simulink model "s_c856m4k_pre_buf"  (R2016b)
(part 3 of 50)

      mask TypeOptions io_dir: To Processor | From Processor
      mask Callback io_dir:
      | mask_enables = get_param(gcb, 'MaskEnables');
      | mask_names = get_param(gcb, 'MaskNames');
      | if strcmp(get_param(gcb, 'io_dir'), 'To Processor'),
      |     mask_enables{ismember(mask_names, 'sample_period')} = 'off';
      | else
      |     mask_enables{ismember(mask_names, 'sample_period')} = 'on';
      | end
      | set_param(gcb, 'MaskEnables', mask_enables);
  spead_valid_err_less : Subsystem  Tag=xps:sw_reg  AncestorBlock=xps_library/software_register  mask(swreg){io_dir=To Processor, io_delay=0, sample_period=1, names=reg, bitwidths=1, bin_pts=0, arith_types=2, sim_port=off, show_format=on}
      mask prompts: io_dir "I/O direction"; io_delay "I/O delay"; sample_period "Sample period"; names "Bitfield names [msb...lsb]"; bitwidths "Bitfield widths"; bin_pts "Bitfield binary pts"; arith_types "Bitfield types, ufix=0, fix=1, bool=2"; sim_port "Provide sim input/output?"; show_format "Print format string?"
      mask help: A 32-bit software-accessible register. Can be divided into bitfields of varying widths and types using the fields in the block mask.
      mask init:
      | swreg_init(gcb)
      settings: AttributesFormatString=1output:b = 1 bits
      mask TypeOptions io_dir: To Processor | From Processor
      mask Callback io_dir:
      | mask_enables = get_param(gcb, 'MaskEnables');
      | mask_names = get_param(gcb, 'MaskNames');
      | if strcmp(get_param(gcb, 'io_dir'), 'To Processor'),
      |     mask_enables{ismember(mask_names, 'sample_period')} = 'off';
      | else
      |     mask_enables{ismember(mask_names, 'sample_period')} = 'on';
      | end
      | set_param(gcb, 'MaskEnables', mask_enables);
  spead_valid_len : Subsystem  Tag=xps:sw_reg  AncestorBlock=xps_library/software_register  mask(swreg){io_dir=To Processor, io_delay=0, sample_period=1, names=reg, bitwidths=1, bin_pts=0, arith_types=2, sim_port=off, show_format=on}
      mask prompts: io_dir "I/O direction"; io_delay "I/O delay"; sample_period "Sample period"; names "Bitfield names [msb...lsb]"; bitwidths "Bitfield widths"; bin_pts "Bitfield binary pts"; arith_types "Bitfield types, ufix=0, fix=1, bool=2"; sim_port "Provide sim input/output?"; show_format "Print format string?"
      mask help: A 32-bit software-accessible register. Can be divided into bitfields of varying widths and types using the fields in the block mask.
      mask init:
      | swreg_init(gcb)
      settings: AttributesFormatString=1output:b = 1 bits
      mask TypeOptions io_dir: To Processor | From Processor
      mask Callback io_dir:
      | mask_enables = get_param(gcb, 'MaskEnables');
      | mask_names = get_param(gcb, 'MaskNames');
      | if strcmp(get_param(gcb, 'io_dir'), 'To Processor'),
      |     mask_enables{ismember(mask_names, 'sample_period')} = 'off';
      | else
      |     mask_enables{ismember(mask_names, 'sample_period')} = 'on';
      | end
      | set_param(gcb, 'MaskEnables', mask_enables);
  spead_valid_len_cnt : Subsystem  Tag=xps:sw_reg  AncestorBlock=xps_library/software_register  mask(swreg){io_dir=To Processor, io_delay=0, sample_period=1, names=reg, bitwidths=32, bin_pts=0, arith_types=0, sim_port=off, show_format=on}
      mask prompts: io_dir "I/O direction"; io_delay "I/O delay"; sample_period "Sample period"; names "Bitfield names [msb...lsb]"; bitwidths "Bitfield widths"; bin_pts "Bitfield binary pts"; arith_types "Bitfield types, ufix=0, fix=1, bool=2"; sim_port "Provide sim input/output?"; show_format "Print format string?"
      mask help: A 32-bit software-accessible register. Can be divided into bitfields of varying widths and types using the fields in the block mask.
      mask init:
      | swreg_init(gcb)
      settings: AttributesFormatString=1output:uf32.0 = 32 bits
      mask TypeOptions io_dir: To Processor | From Processor
      mask Callback io_dir:
      | mask_enables = get_param(gcb, 'MaskEnables');
      | mask_names = get_param(gcb, 'MaskNames');
      | if strcmp(get_param(gcb, 'io_dir'), 'To Processor'),
      |     mask_enables{ismember(mask_names, 'sample_period')} = 'off';
      | else
      |     mask_enables{ismember(mask_names, 'sample_period')} = 'on';
      | end
      | set_param(gcb, 'MaskEnables', mask_enables);
  speadsnap_control : Subsystem  Tag=xps:sw_reg  AncestorBlock=xps_library/software_register  mask(swreg){io_dir=From Processor, io_delay=0, sample_period=1, names=[speadsnap_arm], bitwidths=1, bin_pts=0, arith_types=2, sim_port=off, show_format=on}
      mask prompts: io_dir "I/O direction"; io_delay "I/O delay"; sample_period "Sample period"; names "Bitfield names [msb...lsb]"; bitwidths "Bitfield widths"; bin_pts "Bitfield binary pts"; arith_types "Bitfield types, ufix=0, fix=1, bool=2"; sim_port "Provide sim input/output?"; show_format "Print format string?"
      mask help: A 32-bit software-accessible register. Can be divided into bitfields of varying widths and types using the fields in the block mask.
      mask init:
      | swreg_init(gcb)
      settings: AttributesFormatString=1input:b = 1 bits
      mask TypeOptions io_dir: To Processor | From Processor
      mask Callback io_dir:
      | mask_enables = get_param(gcb, 'MaskEnables');
      | mask_names = get_param(gcb, 'MaskNames');
      | if strcmp(get_param(gcb, 'io_dir'), 'To Processor'),
      |     mask_enables{ismember(mask_names, 'sample_period')} = 'off';
      | else
      |     mask_enables{ismember(mask_names, 'sample_period')} = 'on';
      | end
      | set_param(gcb, 'MaskEnables', mask_enables);
  speadtime0_offset : Subsystem  Tag=xps:sw_reg  AncestorBlock=xps_library/software_register  mask(swreg){io_dir=From Processor, io_delay=1, sample_period=1, names=speadtime_offset0, bitwidths=32, bin_pts=0, arith_types=0, sim_port=on, show_format=on}
      mask prompts: io_dir "I/O direction"; io_delay "I/O delay"; sample_period "Sample period"; names "Bitfield names [msb...lsb]"; bitwidths "Bitfield widths"; bin_pts "Bitfield binary pts"; arith_types "Bitfield types, ufix=0, fix=1, bool=2"; sim_port "Provide sim input/output?"; show_format "Print format string?"
      mask help: A 32-bit software-accessible register. Can be divided into bitfields of varying widths and types using the fields in the block mask.
      mask init:
      | swreg_init(gcb)
      settings: AttributesFormatString=1input:uf32.0 = 32 bits
      mask TypeOptions io_dir: To Processor | From Processor
      mask Callback io_dir:
      | mask_enables = get_param(gcb, 'MaskEnables');
      | mask_names = get_param(gcb, 'MaskNames');
      | if strcmp(get_param(gcb, 'io_dir'), 'To Processor'),
      |     mask_enables{ismember(mask_names, 'sample_period')} = 'off';
      | else
      |     mask_enables{ismember(mask_names, 'sample_period')} = 'on';
      | end
      | set_param(gcb, 'MaskEnables', mask_enables);
  speadtime1_offset : Subsystem  Tag=xps:sw_reg  AncestorBlock=xps_library/software_register  mask(swreg){io_dir=From Processor, io_delay=1, sample_period=1, names=speadtime_offset1, bitwidths=32, bin_pts=0, arith_types=0, sim_port=on, show_format=on}
      mask prompts: io_dir "I/O direction"; io_delay "I/O delay"; sample_period "Sample period"; names "Bitfield names [msb...lsb]"; bitwidths "Bitfield widths"; bin_pts "Bitfield binary pts"; arith_types "Bitfield types, ufix=0, fix=1, bool=2"; sim_port "Provide sim input/output?"; show_format "Print format string?"
      mask help: A 32-bit software-accessible register. Can be divided into bitfields of varying widths and types using the fields in the block mask.
      mask init:
      | swreg_init(gcb)
      settings: AttributesFormatString=1input:uf32.0 = 32 bits
      mask TypeOptions io_dir: To Processor | From Processor
      mask Callback io_dir:
      | mask_enables = get_param(gcb, 'MaskEnables');
      | mask_names = get_param(gcb, 'MaskNames');
      | if strcmp(get_param(gcb, 'io_dir'), 'To Processor'),
      |     mask_enables{ismember(mask_names, 'sample_period')} = 'off';
      | else
      |     mask_enables{ismember(mask_names, 'sample_period')} = 'on';
      | end
      | set_param(gcb, 'MaskEnables', mask_enables);
  src_sel_cntrl : Subsystem  Tag=xps:sw_reg  AncestorBlock=xps_library/software_register  mask(swreg){io_dir=From Processor, io_delay=1, sample_period=1, names=[src_sel_0 src_sel_1], bitwidths=[2 2], bin_pts=[0 0], arith_types=[0 0], sim_port=on, show_format=on}
      mask prompts: io_dir "I/O direction"; io_delay "I/O delay"; sample_period "Sample period"; names "Bitfield names [msb...lsb]"; bitwidths "Bitfield widths"; bin_pts "Bitfield binary pts"; arith_types "Bitfield types, ufix=0, fix=1, bool=2"; sim_port "Provide sim input/output?"; show_format "Print format string?"
      mask help: A 32-bit software-accessible register. Can be divided into bitfields of varying widths and types using the fields in the block mask.
      mask init:
      | swreg_init(gcb)
      settings: AttributesFormatString=2 inputs:uf2.0,uf2.0 = 4 bits
      mask TypeOptions io_dir: To Processor | From Processor
      mask Callback io_dir:
      | mask_enables = get_param(gcb, 'MaskEnables');
      | mask_names = get_param(gcb, 'MaskNames');
      | if strcmp(get_param(gcb, 'io_dir'), 'To Processor'),
      |     mask_enables{ismember(mask_names, 'sample_period')} = 'off';
      | else
      |     mask_enables{ismember(mask_names, 'sample_period')} = 'on';
      | end
      | set_param(gcb, 'MaskEnables', mask_enables);
  ss_cwg0 : Subsystem  Tag=casper:bitsnap  AncestorBlock=casper_library_scopes/bitfield snapshot  mask(bitsnap){io_names=[d0 d1 d2 d3 d4 d5 d6 d7 gpio_trig], io_widths=[10 10 10 10 10 10 10 10 1], io_bps=[9 9 9 9 9 9 9 9 0], io_types=[1 1 1 1 1 1 1 1 2], show_format=on, snap_storage=bram, snap_dram_dimm=2, snap_dram_clock=250, snap_nsamples=11, snap_data_width=128, snap_offset=on, snap_circap=off, snap_value=off, snap_use_dsp48=off, snap_delay=1, extra_names=[c d], extra_widths=[30 2], extra_bps=[0 0], extra_types=[0 0]}
      mask prompts: io_names "Names [msb...lsb]"; io_widths "Bitwidths [msb...lsb]"; io_bps "Binary pts [msb...lsb]"; io_types "Data types [msb...lsb], ufix=0, fix=1, bool=2"; show_format "Print format string?"; snap_storage "Storage medium"; snap_dram_dimm "DRAM dimm"; snap_dram_clock "DRAM clock rate"; snap_nsamples "Number of Samples (2^?)"; snap_data_width "Data width"; snap_offset "Start delay support"; snap_circap "Circular capture support"; snap_value "Extra value capture support"; snap_use_dsp48 "Use DSP48s to implement counters"; snap_delay "Pre-snapshot delay"; extra_names "Names [msb...lsb]"; extra_widths "Widths [msb...lsb]"; extra_bps "Binary pts [msb...lsb]"; extra_types "Data types [msb...lsb], ufix=0, fix=1, bool=2"
      mask help:
      | A wrapped snapshot block. Allows specification of inputs to a snapblock word so the toolflow can automatically set up the scope.
      | See documentation for snapshot for explanation of parameters.
      mask init:
      | bitsnap_init(gcb);
      settings: AttributesFormatString=|
      | snap(9):f10.9,f10.9,f10.9,f10.9,f10.9,f10.9,f10.9,f10.9,b = 81 bits\n128 wide, 2048 deep
      | debugID: 126004058
      mask TypeOptions snap_storage: bram | dram
      mask Callback snap_storage: bitsnap_callback();
      mask TypeOptions snap_dram_dimm: 1 | 2 | 3 | 4
      mask TypeOptions snap_dram_clock: 200 | 250 | 266 | 300 | 333
      mask TypeOptions snap_data_width: 8 | 16 | 32 | 64 | 128
      mask Callback snap_value: bitsnap_callback();
  ss_fifo_in : Subsystem  Tag=casper:bitsnap  AncestorBlock=casper_library_scopes/bitfield snapshot  mask(bitsnap){io_names=[d0 d1 d2 d3 d4 d5 d6 d7 gpio_trig], io_widths=[10 10 10 10 10 10 10 10 1], io_bps=[9 9 9 9 9 9 9 9 0], io_types=[1 1 1 1 1 1 1 1 2], show_format=on, snap_storage=bram, snap_dram_dimm=2, snap_dram_clock=250, snap_nsamples=11, snap_data_width=128, snap_offset=on, snap_circap=off, snap_value=off, snap_use_dsp48=off, snap_delay=1, extra_names=[c d], extra_widths=[30 2], extra_bps=[0 0], extra_types=[0 0]}
      mask prompts: io_names "Names [msb...lsb]"; io_widths "Bitwidths [msb...lsb]"; io_bps "Binary pts [msb...lsb]"; io_types "Data types [msb...lsb], ufix=0, fix=1, bool=2"; show_format "Print format string?"; snap_storage "Storage medium"; snap_dram_dimm "DRAM dimm"; snap_dram_clock "DRAM clock rate"; snap_nsamples "Number of Samples (2^?)"; snap_data_width "Data width"; snap_offset "Start delay support"; snap_circap "Circular capture support"; snap_value "Extra value capture support"; snap_use_dsp48 "Use DSP48s to implement counters"; snap_delay "Pre-snapshot delay"; extra_names "Names [msb...lsb]"; extra_widths "Widths [msb...lsb]"; extra_bps "Binary pts [msb...lsb]"; extra_types "Data types [msb...lsb], ufix=0, fix=1, bool=2"
      mask help:
      | A wrapped snapshot block. Allows specification of inputs to a snapblock word so the toolflow can automatically set up the scope.
      | See documentation for snapshot for explanation of parameters.
      mask init:
      | bitsnap_init(gcb);
      settings: AttributesFormatString=|
      | snap(9):f10.9,f10.9,f10.9,f10.9,f10.9,f10.9,f10.9,f10.9,b = 81 bits\n128 wide, 2048 deep
      | debugID: 107099023
      mask TypeOptions snap_storage: bram | dram
      mask Callback snap_storage: bitsnap_callback();
      mask TypeOptions snap_dram_dimm: 1 | 2 | 3 | 4
      mask TypeOptions snap_dram_clock: 200 | 250 | 266 | 300 | 333
      mask TypeOptions snap_data_width: 8 | 16 | 32 | 64 | 128
      mask Callback snap_value: bitsnap_callback();
  ss_localtime : Subsystem  Tag=casper:bitsnap  AncestorBlock=casper_library_scopes/bitfield snapshot  mask(bitsnap){io_names=time, io_widths=64, io_bps=0, io_types=0, show_format=on, snap_storage=bram, snap_dram_dimm=2, snap_dram_clock=250, snap_nsamples=11, snap_data_width=64, snap_offset=on, snap_circap=off, snap_value=off, snap_use_dsp48=off, snap_delay=1, extra_names=[c d], extra_widths=[30 2], extra_bps=[0 0], extra_types=[0 0]}
      mask prompts: io_names "Names [msb...lsb]"; io_widths "Bitwidths [msb...lsb]"; io_bps "Binary pts [msb...lsb]"; io_types "Data types [msb...lsb], ufix=0, fix=1, bool=2"; show_format "Print format string?"; snap_storage "Storage medium"; snap_dram_dimm "DRAM dimm"; snap_dram_clock "DRAM clock rate"; snap_nsamples "Number of Samples (2^?)"; snap_data_width "Data width"; snap_offset "Start delay support"; snap_circap "Circular capture support"; snap_value "Extra value capture support"; snap_use_dsp48 "Use DSP48s to implement counters"; snap_delay "Pre-snapshot delay"; extra_names "Names [msb...lsb]"; extra_widths "Widths [msb...lsb]"; extra_bps "Binary pts [msb...lsb]"; extra_types "Data types [msb...lsb], ufix=0, fix=1, bool=2"
      mask help:
      | A wrapped snapshot block. Allows specification of inputs to a snapblock word so the toolflow can automatically set up the scope.
      | See documentation for snapshot for explanation of parameters.
      mask init:
      | bitsnap_init(gcb);
      settings: AttributesFormatString=|
      | snap(1):uf64.0 = 64 bits\n64 wide, 2048 deep
      | debugID: 12399183
      mask TypeOptions snap_storage: bram | dram
      mask Callback snap_storage: bitsnap_callback();
      mask TypeOptions snap_dram_dimm: 1 | 2 | 3 | 4
      mask TypeOptions snap_dram_clock: 200 | 250 | 266 | 300 | 333
      mask TypeOptions snap_data_width: 8 | 16 | 32 | 64 | 128
      mask Callback snap_value: bitsnap_callback();
  ss_trig_time_lsw : Subsystem  Tag=xps:sw_reg  AncestorBlock=xps_library/software_register  mask(swreg){io_dir=From Processor, io_delay=1, sample_period=1, names=reg, bitwidths=32, bin_pts=0, arith_types=0, sim_port=on, show_format=on}
      mask prompts: io_dir "I/O direction"; io_delay "I/O delay"; sample_period "Sample period"; names "Bitfield names [msb...lsb]"; bitwidths "Bitfield widths"; bin_pts "Bitfield binary pts"; arith_types "Bitfield types, ufix=0, fix=1, bool=2"; sim_port "Provide sim input/output?"; show_format "Print format string?"
      mask help: A 32-bit software-accessible register. Can be divided into bitfields of varying widths and types using the fields in the block mask.
      mask init:
      | swreg_init(gcb)
      settings: AttributesFormatString=1input:uf32.0 = 32 bits
      mask TypeOptions io_dir: To Processor | From Processor
      mask Callback io_dir:
      | mask_enables = get_param(gcb, 'MaskEnables');
      | mask_names = get_param(gcb, 'MaskNames');
      | if strcmp(get_param(gcb, 'io_dir'), 'To Processor'),
      |     mask_enables{ismember(mask_names, 'sample_period')} = 'off';
      | else
      |     mask_enables{ismember(mask_names, 'sample_period')} = 'on';
      | end
      | set_param(gcb, 'MaskEnables', mask_enables);
  ss_trig_time_msw : Subsystem  Tag=xps:sw_reg  AncestorBlock=xps_library/software_register  mask(swreg){io_dir=From Processor, io_delay=1, sample_period=1, names=reg, bitwidths=32, bin_pts=0, arith_types=0, sim_port=on, show_format=on}
      mask prompts: io_dir "I/O direction"; io_delay "I/O delay"; sample_period "Sample period"; names "Bitfield names [msb...lsb]"; bitwidths "Bitfield widths"; bin_pts "Bitfield binary pts"; arith_types "Bitfield types, ufix=0, fix=1, bool=2"; sim_port "Provide sim input/output?"; show_format "Print format string?"
      mask help: A 32-bit software-accessible register. Can be divided into bitfields of varying widths and types using the fields in the block mask.
      mask init:
      | swreg_init(gcb)
      settings: AttributesFormatString=1input:uf32.0 = 32 bits
      mask TypeOptions io_dir: To Processor | From Processor
      mask Callback io_dir:
      | mask_enables = get_param(gcb, 'MaskEnables');
      | mask_names = get_param(gcb, 'MaskNames');
      | if strcmp(get_param(gcb, 'io_dir'), 'To Processor'),
      |     mask_enables{ismember(mask_names, 'sample_period')} = 'off';
      | else
      |     mask_enables{ismember(mask_names, 'sample_period')} = 'on';
      | end
      | set_param(gcb, 'MaskEnables', mask_enables);
  start_flag_lsw : Subsystem  Tag=xps:sw_reg  AncestorBlock=xps_library/software_register  mask(swreg){io_dir=From Processor, io_delay=1, sample_period=1, names=reg, bitwidths=32, bin_pts=0, arith_types=0, sim_port=on, show_format=on}
      mask prompts: io_dir "I/O direction"; io_delay "I/O delay"; sample_period "Sample period"; names "Bitfield names [msb...lsb]"; bitwidths "Bitfield widths"; bin_pts "Bitfield binary pts"; arith_types "Bitfield types, ufix=0, fix=1, bool=2"; sim_port "Provide sim input/output?"; show_format "Print format string?"
      mask help: A 32-bit software-accessible register. Can be divided into bitfields of varying widths and types using the fields in the block mask.
      mask init:
      | swreg_init(gcb)
      settings: AttributesFormatString=1input:uf32.0 = 32 bits
      mask TypeOptions io_dir: To Processor | From Processor
      mask Callback io_dir:
      | mask_enables = get_param(gcb, 'MaskEnables');
      | mask_names = get_param(gcb, 'MaskNames');
      | if strcmp(get_param(gcb, 'io_dir'), 'To Processor'),
      |     mask_enables{ismember(mask_names, 'sample_period')} = 'off';
      | else
      |     mask_enables{ismember(mask_names, 'sample_period')} = 'on';
      | end
      | set_param(gcb, 'MaskEnables', mask_enables);
  start_flag_msw : Subsystem  Tag=xps:sw_reg  AncestorBlock=xps_library/software_register  mask(swreg){io_dir=From Processor, io_delay=1, sample_period=1, names=reg, bitwidths=32, bin_pts=0, arith_types=0, sim_port=on, show_format=on}
      mask prompts: io_dir "I/O direction"; io_delay "I/O delay"; sample_period "Sample period"; names "Bitfield names [msb...lsb]"; bitwidths "Bitfield widths"; bin_pts "Bitfield binary pts"; arith_types "Bitfield types, ufix=0, fix=1, bool=2"; sim_port "Provide sim input/output?"; show_format "Print format string?"
      mask help: A 32-bit software-accessible register. Can be divided into bitfields of varying widths and types using the fields in the block mask.
      mask init:
      | swreg_init(gcb)
      settings: AttributesFormatString=1input:uf32.0 = 32 bits
      mask TypeOptions io_dir: To Processor | From Processor
      mask Callback io_dir:
      | mask_enables = get_param(gcb, 'MaskEnables');
      | mask_names = get_param(gcb, 'MaskNames');
      | if strcmp(get_param(gcb, 'io_dir'), 'To Processor'),
      |     mask_enables{ismember(mask_names, 'sample_period')} = 'off';
      | else
      |     mask_enables{ismember(mask_names, 'sample_period')} = 'on';
      | end
      | set_param(gcb, 'MaskEnables', mask_enables);
  start_load_time_lsw : Subsystem  Tag=xps:sw_reg  AncestorBlock=xps_library/software_register  mask(swreg){io_dir=From Processor, io_delay=1, sample_period=1, names=reg, bitwidths=32, bin_pts=0, arith_types=0, sim_port=on, show_format=on}
      mask prompts: io_dir "I/O direction"; io_delay "I/O delay"; sample_period "Sample period"; names "Bitfield names [msb...lsb]"; bitwidths "Bitfield widths"; bin_pts "Bitfield binary pts"; arith_types "Bitfield types, ufix=0, fix=1, bool=2"; sim_port "Provide sim input/output?"; show_format "Print format string?"
      mask help: A 32-bit software-accessible register. Can be divided into bitfields of varying widths and types using the fields in the block mask.
      mask init:
      | swreg_init(gcb)
      settings: AttributesFormatString=1input:uf32.0 = 32 bits
      mask TypeOptions io_dir: To Processor | From Processor
      mask Callback io_dir:
      | mask_enables = get_param(gcb, 'MaskEnables');
      | mask_names = get_param(gcb, 'MaskNames');
      | if strcmp(get_param(gcb, 'io_dir'), 'To Processor'),
      |     mask_enables{ismember(mask_names, 'sample_period')} = 'off';
      | else
      |     mask_enables{ismember(mask_names, 'sample_period')} = 'on';
      | end
      | set_param(gcb, 'MaskEnables', mask_enables);
  start_load_time_msw : Subsystem  Tag=xps:sw_reg  AncestorBlock=xps_library/software_register  mask(swreg){io_dir=From Processor, io_delay=1, sample_period=1, names=reg, bitwidths=32, bin_pts=0, arith_types=0, sim_port=on, show_format=on}
      mask prompts: io_dir "I/O direction"; io_delay "I/O delay"; sample_period "Sample period"; names "Bitfield names [msb...lsb]"; bitwidths "Bitfield widths"; bin_pts "Bitfield binary pts"; arith_types "Bitfield types, ufix=0, fix=1, bool=2"; sim_port "Provide sim input/output?"; show_format "Print format string?"
      mask help: A 32-bit software-accessible register. Can be divided into bitfields of varying widths and types using the fields in the block mask.
      mask init:
      | swreg_init(gcb)
      settings: AttributesFormatString=1input:uf32.0 = 32 bits
      mask TypeOptions io_dir: To Processor | From Processor
      mask Callback io_dir:
      | mask_enables = get_param(gcb, 'MaskEnables');
      | mask_names = get_param(gcb, 'MaskNames');
      | if strcmp(get_param(gcb, 'io_dir'), 'To Processor'),
      |     mask_enables{ismember(mask_names, 'sample_period')} = 'off';
      | else
      |     mask_enables{ismember(mask_names, 'sample_period')} = 'on';
      | end
      | set_param(gcb, 'MaskEnables', mask_enables);
  start_time_lsw : Subsystem  Tag=xps:sw_reg  AncestorBlock=xps_library/software_register  mask(swreg){io_dir=From Processor, io_delay=1, sample_period=1, names=reg, bitwidths=32, bin_pts=0, arith_types=0, sim_port=on, show_format=on}
      mask prompts: io_dir "I/O direction"; io_delay "I/O delay"; sample_period "Sample period"; names "Bitfield names [msb...lsb]"; bitwidths "Bitfield widths"; bin_pts "Bitfield binary pts"; arith_types "Bitfield types, ufix=0, fix=1, bool=2"; sim_port "Provide sim input/output?"; show_format "Print format string?"
      mask help: A 32-bit software-accessible register. Can be divided into bitfields of varying widths and types using the fields in the block mask.
      mask init:
      | swreg_init(gcb)
      settings: AttributesFormatString=1input:uf32.0 = 32 bits
      mask TypeOptions io_dir: To Processor | From Processor
      mask Callback io_dir:
      | mask_enables = get_param(gcb, 'MaskEnables');
      | mask_names = get_param(gcb, 'MaskNames');
      | if strcmp(get_param(gcb, 'io_dir'), 'To Processor'),
      |     mask_enables{ismember(mask_names, 'sample_period')} = 'off';
      | else
      |     mask_enables{ismember(mask_names, 'sample_period')} = 'on';
      | end
      | set_param(gcb, 'MaskEnables', mask_enables);
  start_time_msw : Subsystem  Tag=xps:sw_reg  AncestorBlock=xps_library/software_register  mask(swreg){io_dir=From Processor, io_delay=1, sample_period=1, names=reg, bitwidths=32, bin_pts=0, arith_types=0, sim_port=on, show_format=on}
      mask prompts: io_dir "I/O direction"; io_delay "I/O delay"; sample_period "Sample period"; names "Bitfield names [msb...lsb]"; bitwidths "Bitfield widths"; bin_pts "Bitfield binary pts"; arith_types "Bitfield types, ufix=0, fix=1, bool=2"; sim_port "Provide sim input/output?"; show_format "Print format string?"
      mask help: A 32-bit software-accessible register. Can be divided into bitfields of varying widths and types using the fields in the block mask.
      mask init:
      | swreg_init(gcb)
      settings: AttributesFormatString=1input:uf32.0 = 32 bits
      mask TypeOptions io_dir: To Processor | From Processor
      mask Callback io_dir:
      | mask_enables = get_param(gcb, 'MaskEnables');
      | mask_names = get_param(gcb, 'MaskNames');
      | if strcmp(get_param(gcb, 'io_dir'), 'To Processor'),
      |     mask_enables{ismember(mask_names, 'sample_period')} = 'off';
      | else
      |     mask_enables{ismember(mask_names, 'sample_period')} = 'on';
      | end
      | set_param(gcb, 'MaskEnables', mask_enables);
  status0 : Subsystem  Tag=xps:sw_reg  AncestorBlock=xps_library/software_register  mask(swreg){io_dir=To Processor, io_delay=0, sample_period=1, names=[led_up led_rx led_tx tx_afull tx_overflow rx_overrun], bitwidths=1, bin_pts=0, arith_types=2, sim_port=off, show_format=on}
      mask prompts: io_dir "I/O direction"; io_delay "I/O delay"; sample_period "Sample period"; names "Bitfield names [msb...lsb]"; bitwidths "Bitfield widths"; bin_pts "Bitfield binary pts"; arith_types "Bitfield types, ufix=0, fix=1, bool=2"; sim_port "Provide sim input/output?"; show_format "Print format string?"
      mask help: A 32-bit software-accessible register. Can be divided into bitfields of varying widths and types using the fields in the block mask.
      mask init:
      | swreg_init(gcb)
      settings: AttributesFormatString=6 outputs:b,b,b,b,b,b = 6 bits
      mask TypeOptions io_dir: To Processor | From Processor
      mask Callback io_dir:
      | mask_enables = get_param(gcb, 'MaskEnables');
      | mask_names = get_param(gcb, 'MaskNames');
      | if strcmp(get_param(gcb, 'io_dir'), 'To Processor'),
      |     mask_enables{ismember(mask_names, 'sample_period')} = 'off';
      | else
      |     mask_enables{ismember(mask_names, 'sample_period')} = 'on';
      | end
      | set_param(gcb, 'MaskEnables', mask_enables);
  stop_load_time_lsw : Subsystem  Tag=xps:sw_reg  AncestorBlock=xps_library/software_register  mask(swreg){io_dir=From Processor, io_delay=1, sample_period=1, names=reg, bitwidths=32, bin_pts=0, arith_types=0, sim_port=on, show_format=on}
      mask prompts: io_dir "I/O direction"; io_delay "I/O delay"; sample_period "Sample period"; names "Bitfield names [msb...lsb]"; bitwidths "Bitfield widths"; bin_pts "Bitfield binary pts"; arith_types "Bitfield types, ufix=0, fix=1, bool=2"; sim_port "Provide sim input/output?"; show_format "Print format string?"
      mask help: A 32-bit software-accessible register. Can be divided into bitfields of varying widths and types using the fields in the block mask.
      mask init:
      | swreg_init(gcb)
      settings: AttributesFormatString=1input:uf32.0 = 32 bits
      mask TypeOptions io_dir: To Processor | From Processor
      mask Callback io_dir:
      | mask_enables = get_param(gcb, 'MaskEnables');
      | mask_names = get_param(gcb, 'MaskNames');
      | if strcmp(get_param(gcb, 'io_dir'), 'To Processor'),
      |     mask_enables{ismember(mask_names, 'sample_period')} = 'off';
      | else
      |     mask_enables{ismember(mask_names, 'sample_period')} = 'on';
      | end
      | set_param(gcb, 'MaskEnables', mask_enables);
  stop_load_time_msw : Subsystem  Tag=xps:sw_reg  AncestorBlock=xps_library/software_register  mask(swreg){io_dir=From Processor, io_delay=1, sample_period=1, names=reg, bitwidths=32, bin_pts=0, arith_types=0, sim_port=on, show_format=on}
      mask prompts: io_dir "I/O direction"; io_delay "I/O delay"; sample_period "Sample period"; names "Bitfield names [msb...lsb]"; bitwidths "Bitfield widths"; bin_pts "Bitfield binary pts"; arith_types "Bitfield types, ufix=0, fix=1, bool=2"; sim_port "Provide sim input/output?"; show_format "Print format string?"
      mask help: A 32-bit software-accessible register. Can be divided into bitfields of varying widths and types using the fields in the block mask.
      mask init:
      | swreg_init(gcb)
      settings: AttributesFormatString=1input:uf32.0 = 32 bits
      mask TypeOptions io_dir: To Processor | From Processor
      mask Callback io_dir:
      | mask_enables = get_param(gcb, 'MaskEnables');
      | mask_names = get_param(gcb, 'MaskNames');
      | if strcmp(get_param(gcb, 'io_dir'), 'To Processor'),
      |     mask_enables{ismember(mask_names, 'sample_period')} = 'off';
      | else
      |     mask_enables{ismember(mask_names, 'sample_period')} = 'on';
      | end
      | set_param(gcb, 'MaskEnables', mask_enables);
  test_control : Subsystem  Tag=xps:sw_reg  AncestorBlock=xps_library/software_register  mask(swreg){io_dir=From Processor, io_delay=0, sample_period=1, names=[sel_ramp80 rst_ramp80], bitwidths=1, bin_pts=0, arith_types=2, sim_port=on, show_format=on}
      mask prompts: io_dir "I/O direction"; io_delay "I/O delay"; sample_period "Sample period"; names "Bitfield names [msb...lsb]"; bitwidths "Bitfield widths"; bin_pts "Bitfield binary pts"; arith_types "Bitfield types, ufix=0, fix=1, bool=2"; sim_port "Provide sim input/output?"; show_format "Print format string?"
      mask help: A 32-bit software-accessible register. Can be divided into bitfields of varying widths and types using the fields in the block mask.
      mask init:
      | swreg_init(gcb)
      settings: AttributesFormatString=2 inputs:b,b = 2 bits
      mask TypeOptions io_dir: To Processor | From Processor
      mask Callback io_dir:
      | mask_enables = get_param(gcb, 'MaskEnables');
      | mask_names = get_param(gcb, 'MaskNames');
      | if strcmp(get_param(gcb, 'io_dir'), 'To Processor'),
      |     mask_enables{ismember(mask_names, 'sample_period')} = 'off';
      | else
      |     mask_enables{ismember(mask_names, 'sample_period')} = 'on';
      | end
      | set_param(gcb, 'MaskEnables', mask_enables);
  tick_offset_lsw : Subsystem  Tag=xps:sw_reg  AncestorBlock=xps_library/software_register  mask(swreg){io_dir=From Processor, io_delay=1, sample_period=1, names=reg, bitwidths=32, bin_pts=0, arith_types=0, sim_port=on, show_format=on}
      mask prompts: io_dir "I/O direction"; io_delay "I/O delay"; sample_period "Sample period"; names "Bitfield names [msb...lsb]"; bitwidths "Bitfield widths"; bin_pts "Bitfield binary pts"; arith_types "Bitfield types, ufix=0, fix=1, bool=2"; sim_port "Provide sim input/output?"; show_format "Print format string?"
      mask help: A 32-bit software-accessible register. Can be divided into bitfields of varying widths and types using the fields in the block mask.
      mask init:
      | swreg_init(gcb)
      settings: AttributesFormatString=1input:uf32.0 = 32 bits
      mask TypeOptions io_dir: To Processor | From Processor
      mask Callback io_dir:
      | mask_enables = get_param(gcb, 'MaskEnables');
      | mask_names = get_param(gcb, 'MaskNames');
      | if strcmp(get_param(gcb, 'io_dir'), 'To Processor'),
      |     mask_enables{ismember(mask_names, 'sample_period')} = 'off';
      | else
      |     mask_enables{ismember(mask_names, 'sample_period')} = 'on';
      | end
      | set_param(gcb, 'MaskEnables', mask_enables);
  tick_offset_msw : Subsystem  Tag=xps:sw_reg  AncestorBlock=xps_library/software_register  mask(swreg){io_dir=From Processor, io_delay=1, sample_period=1, names=reg, bitwidths=32, bin_pts=0, arith_types=0, sim_port=on, show_format=on}
      mask prompts: io_dir "I/O direction"; io_delay "I/O delay"; sample_period "Sample period"; names "Bitfield names [msb...lsb]"; bitwidths "Bitfield widths"; bin_pts "Bitfield binary pts"; arith_types "Bitfield types, ufix=0, fix=1, bool=2"; sim_port "Provide sim input/output?"; show_format "Print format string?"
      mask help: A 32-bit software-accessible register. Can be divided into bitfields of varying widths and types using the fields in the block mask.
      mask init:
      | swreg_init(gcb)
      settings: AttributesFormatString=1input:uf32.0 = 32 bits
      mask TypeOptions io_dir: To Processor | From Processor
      mask Callback io_dir:
      | mask_enables = get_param(gcb, 'MaskEnables');
      | mask_names = get_param(gcb, 'MaskNames');
      | if strcmp(get_param(gcb, 'io_dir'), 'To Processor'),
      |     mask_enables{ismember(mask_names, 'sample_period')} = 'off';
      | else
      |     mask_enables{ismember(mask_names, 'sample_period')} = 'on';
      | end
      | set_param(gcb, 'MaskEnables', mask_enables);
  ticks_since_mrst : Subsystem
  tvg_spead_time_with_pkt_ctr : Subsystem  mask{packetlen_bits=9}
      mask prompts: packetlen_bits "Packet length, num 80-bit words (2^?):"
  wng0 : Subsystem
  wng_corr : Subsystem
  wng_rst : Subsystem
  wr_addr{0..3} (4 alike) : xbsIndex_r4/Counter  cnt_type=Free Running  cnt_to=Inf  operation=Up  start_count=0  cnt_by_val=1  arith_type=Unsigned  n_bits=10  bin_pt=0  load_pin=off  rst=on  en=on  explicit_period=on  period=1  use_behavioral_HDL=off  implementation=Fabric  dbl_ovrd=off  block_type=counter
  tag scope: arb_en0=global, arb_rst0=global, cnt_rst=global, dram_addr_offset0=global, dram_rd_repeat0=global, dram_rd_repeat_delay0=global, dram_rd_trig0=global, dram_read_length0=global, dram_tvg0=global, dram_tvg_length0=global, local_time=global, tvg_sel0=global
  wires:
  gbe_porttx/1(in_reg) -> pipeline242/1(d)
  Constant197/1 -> gbe_porttx/1(sim_1)
  Constant75/1 -> gbe_iptx0/1(sim_1)
  Constant77/1 -> gbe_iptx1/1(sim_1)
  Constant78/1 -> gbe_iptx2/1(sim_1)
  Constant79/1 -> gbe_iptx3/1(sim_1)
  Constant80/1 -> digitiser_id/1(sim_1)
  Constant82/1 -> receptor_id/1(sim_1)
  Constant81/1 -> digitiser_id/2(sim_2)
  receptor_id/1(in_receptor_id) -> bus_create1/3(in3)
  Constant165/1 -> receptor_id/2(sim_2)
  Constant84/1 -> receptor_id/3(sim_3)
  [masked_time] -> Delay128/1
  tvg_spead_time_with_pkt_ctr/1(local_time) -> Delay131/1
  tvg_spead_time_with_pkt_ctr/3(tvg_data_pol0) -> Delay133/1
  tvg_spead_time_with_pkt_ctr/4(tvg_data_pol1) -> Delay134/1
  tvg_spead_time_with_pkt_ctr/2(spead_time) -> Delay132/1
  [fifoselect] -> edge_detect37/1(in), Inverter2/1
  Register5/1 -> [speadtime0]  "speadtime0"
  Inverter2/1 -> edge_detect38/1(in)
  edge_detect37/1(out) -> Register5/2
  edge_detect38/1(out) -> Register6/2
  Register6/1 -> [speadtime1]  "speadtime1"
  [mrst] -> ticks_since_mrst/1(reset)
  [sync] -> ticks_since_mrst/2(sync)
  ticks_since_mrst/1(time64) -> [local_time]  "localtime"
  [msync] -> [sync]  "sync"
  edge_detect20/1(out) -> [mrst]  "mrst"
  edge_detect6/1(out) -> [msync]  "msync"
  edge_detect36/1(out) -> Terminator83/1  "clr_status"
  [local_time] -> slice1/1, slice2/1
  Constant92/1 -> orig_control/3(sim_3)
  Constant149/1 -> orig_control/1(sim_1)
  Constant90/1 -> orig_control/2(sim_2)
  Constant98/1 -> orig_control/6(sim_6)
  Constant95/1 -> orig_control/5(sim_5)
  Constant124/1 -> orig_control/4(sim_4)
  Pulse Generator/1 -> orig_control/8(sim_8)
  [tick_offset] -> ticks_since_mrst/3(offset)
  edge_detect7/1(out) -> [load_tick_offset]  "mrst"
  Constant86/1 -> orig_control/9(sim_9)
  digitiser_id/1(in_digitiser_serial) -> bus_create1/1(in1)
  digitiser_id/2(in_digitiser_type) -> bus_create1/2(in2)
  Constant148/1 -> flag_setup/3(sim_3)
  Constant147/1 -> flag_setup/2(sim_2)
  Constant143/1 -> flag_setup/1(sim_1)
  Counter Free-Running3/1 -> Relational Operator4/2
  Constant152/1 -> Relational Operator4/1
  Relational Operator4/1 -> flag_setup/4(sim_4)
  Constant157/1 -> start_flag_msw/1(sim_1)
  Constant158/1 -> start_flag_lsw/1(sim_1)
  Constant156/1 -> end_flag_msw/1(sim_1)
  Constant155/1 -> end_flag_lsw/1(sim_1)
  Concat18/1 -> Delay83/1  "starttime"
  Concat19/1 -> Delay85/1  "stoptime"
  [flag_start_time] -> Delay80/1
  [local_time] -> Delay79/1, Delay81/1
  [flag_end_time] -> Delay82/1, Delay86/1
  Relational4/1 -> Logical24/2  "start_okay"
  [flag_armed] -> Delay78/1
  Relational5/1 -> Logical42/2  "end_okay"
  Logical24/1 -> Delay55/1  "start_okay"
  Logical42/1 -> Logical35/1  "end_okay"
  edge_detect41/1(out) -> [load_flag_time]  "loadtimes"
  Constant144/1 -> Register1/1
  edge_detect40/1(out) -> [reset_flag_time]  "rst"
  [reset_flag_time] -> Register1/2
  [load_flag_time] -> Register1/3
  Register1/1 -> [flag_armed]  "armed"
  Relational Operator3/1 -> flag_setup/5(sim_5)
  Relational8/1 -> Delay54/1  "zero_stop"
  Constant85/1 -> Relational8/2
  Logical35/1 -> Logical4/2  "eokay"
  Counter Free-Running2/1 -> Relational Operator3/2
  Constant154/1 -> Relational Operator3/1
  Logical43/1 -> sample_masking/2(den_in)
  Constant153/1 -> start_time_msw/1(sim_1)
  Constant159/1 -> start_time_lsw/1(sim_1)
  Constant94/1 -> end_time_msw/1(sim_1)
  Constant76/1 -> end_time_lsw/1(sim_1)
  Relational9/1 -> Logical44/2  "start_okay"
  Relational17/1 -> Logical46/2  "end_okay"
  [start_time] -> Delay72/1
  Relational19/1 -> Delay40/1  "first_sample"
  [end_time] -> Delay75/1
  Relational20/1 -> Delay41/1  "last_sample"
  [sample_end] -> sample_masking/6(sample_end)
  [sample_start] -> sample_masking/5(sample_start)
  sample_masking/2(den_out) -> Delay126/1  "enable"
  sample_masking/3(data_mask) -> Delay127/1  "mask"
  edge_detect11/1(out) -> [reset_en_time]  "reset_en_time"
  Relational Operator5/1 -> control_output/2(sim_2)
  Counter Free-Running4/1 -> Relational Operator6/2, Relational Operator5/2
  Constant142/1 -> Relational Operator5/1
  edge_detect12/1(out) -> [load_en_time]  "load_en_time"
  Concat10/1 -> Delay76/1
  Concat11/1 -> Delay77/1
  Constant88/1 -> Register2/1
  [reset_en_time] -> Register2/2
  [load_en_time] -> Register2/3
  Register2/1 -> [en_armed]  "armed"
  Logical44/1 -> Delay42/1  "start_okay"
  Logical46/1 -> Logical45/1  "end_okay"
  Logical45/1 -> Logical43/2
  Constant99/1 -> Delay70/1
  Relational18/1 -> Delay39/1
  Constant93/1 -> control_output/3(sim_3)
  Constant151/1 -> control_output/4(sim_4)
  Constant96/1 -> Relational Operator6/1
  Relational Operator6/1 -> control_output/1(sim_1)
  [data_enable] -> Delay129/1
  [sample_mask] -> Delay130/1
  Constant150/1 -> tick_offset_msw/1(sim_1)
  Constant176/1 -> tick_offset_lsw/1(sim_1)
  Concat16/1 -> Register3/1
  [load_tick_offset] -> Register3/2
  Register3/1 -> [tick_offset]
  wng0/1(bus_out) -> [wng0_tp0], pipeline443/1(d)
  bus_addsub/1(dout) -> Delay105/1
  bus_addsub2/1(dout) -> Delay95/1
  bus_addsub4/1(dout) -> bus_convert6/1(din)
  bus_mult/1(a*b) -> [cwg0_tp1], bus_convert/1(din)
  Constant123/1 -> scale_wng0/1(sim_1)
  Constant74/1 -> scale_wng_corr/1(sim_1)
  pipeline309/1(q) -> edge_detect12/1(in)
  pipeline320/1(q) -> edge_detect11/1(in)
  pipeline331/1(q) -> [sample_start]
  pipeline339/1(q) -> [sample_end]
  Delay76/1 -> [start_time]
  Delay77/1 -> [end_time]
  Delay83/1 -> [flag_start_time]
  Delay85/1 -> [flag_end_time]
  pipeline407/1(q) -> wng0/1(scale_16_14)
  pipeline206/1(q) -> [gbe_ip3]
  pipeline212/1(q) -> [gbe_ip2]
  pipeline220/1(q) -> [gbe_ip0]
  Delay126/1 -> [data_enable]
  Delay127/1 -> [sample_mask]
  Delay128/1 -> tvg_spead_time_with_pkt_ctr/1(localtime64)
  Delay129/1 -> tvg_spead_time_with_pkt_ctr/2(data_enable)
  Delay130/1 -> tvg_spead_time_with_pkt_ctr/3(data_mask)
  Delay131/1 -> [tvg_ltime]
  Delay132/1 -> [tvg_stime]
  Delay133/1 -> [tvg_pol0]
  Delay134/1 -> [tvg_pol1]
  Delay105/1 -> bus_convert2/1(din)
  Delay95/1 -> bus_convert4/1(din)
  Delay139/1 -> bus_addsub4/1(a)
  pipeline350/1(q) -> Concat10/1
  pipeline361/1(q) -> Concat10/2
  pipeline372/1(q) -> Concat11/1
  pipeline383/1(q) -> Concat11/2
  pipeline393/1(q) -> [hdr_0x3101]
  pipeline395/1(q) -> [pol0_id]
  pipeline396/1(q) -> [pol1_id]
  orig_control/1(in_up_cnt_rst) -> pipeline204/1(d)
  pipeline204/1(q) -> edge_detect31/1(in)
  orig_control/2(in_tvg_select0) -> pipeline205/1(d)
  orig_control/3(in_tvg_select1) -> pipeline297/1(d)
  orig_control/4(in_clr_status) -> pipeline394/1(d)
  orig_control/5(in_gbe_rst) -> pipeline405/1(d)
  orig_control/6(in_gbe_txen) -> pipeline416/1(d)
  orig_control/7(in_msync) -> pipeline424/1(d)
  orig_control/8(in_mrst) -> pipeline434/1(d)
  orig_control/9(in_load_tick_offset) -> pipeline445/1(d)
  pipeline445/1(q) -> edge_detect7/1(in)
  pipeline434/1(q) -> edge_detect20/1(in)
  pipeline424/1(q) -> edge_detect6/1(in)
  pipeline405/1(q) -> Terminator82/1
  pipeline394/1(q) -> edge_detect36/1(in)
  pipeline297/1(q) -> [tvg_select1]
  pipeline205/1(q) -> [tvg_select0]
  pipeline213/1(q) -> [gbe_ip1]
  gbe_iptx0/1(in_reg) -> pipeline220/1(d)
  gbe_iptx1/1(in_reg) -> pipeline213/1(d)
  gbe_iptx2/1(in_reg) -> pipeline212/1(d)
  gbe_iptx3/1(in_reg) -> pipeline206/1(d)
  tick_offset_msw/1(in_reg) -> pipeline264/1(d)
  pipeline264/1(q) -> Concat16/1
  tick_offset_lsw/1(in_reg) -> pipeline275/1(d)
  pipeline275/1(q) -> Concat16/2
  slice1/1 -> pipeline298/1(d)
  pipeline298/1(q) -> local_time_lsw1/1(out_reg)
  slice2/1 -> pipeline286/1(d)
  pipeline286/1(q) -> local_time_msw1/1(out_reg)
  end_time_lsw/1(in_reg) -> pipeline383/1(d)
  end_time_msw/1(in_reg) -> pipeline372/1(d)
  start_time_lsw/1(in_reg) -> pipeline361/1(d)
  start_time_msw/1(in_reg) -> pipeline350/1(d)
  control_output/4(in_sample_end) -> pipeline339/1(d)
  control_output/3(in_sample_start) -> pipeline331/1(d)
  control_output/2(in_reset_en_time) -> pipeline320/1(d)
  control_output/1(in_load_en_time) -> pipeline309/1(d)
  bus_create1/1(bus_out) -> pipeline393/1(d)
  receptor_id/2(in_pol0_id) -> pipeline395/1(d)
  receptor_id/3(in_pol1_id) -> pipeline396/1(d)
  flag_setup/1(in_adc_count) -> pipeline397/1(d)
  flag_setup/2(in_adc_flag) -> pipeline398/1(d)
  flag_setup/3(in_ndiode_flag) -> pipeline399/1(d)
  flag_setup/4(in_load_flags) -> pipeline400/1(d)
  flag_setup/5(in_reset_flags) -> pipeline401/1(d)
  pipeline401/1(q) -> edge_detect40/1(in)
  pipeline400/1(q) -> edge_detect41/1(in)
  pipeline399/1(q) -> [ndiode_flag]
  pipeline398/1(q) -> [adc_flag]
  pipeline397/1(q) -> [adc_count]
  start_flag_msw/1(in_reg) -> pipeline402/1(d)
  pipeline402/1(q) -> Concat18/1
  start_flag_lsw/1(in_reg) -> pipeline403/1(d)
  pipeline403/1(q) -> Concat18/2
  end_flag_msw/1(in_reg) -> pipeline404/1(d)
  pipeline404/1(q) -> Concat19/1
  end_flag_lsw/1(in_reg) -> pipeline406/1(d)
  pipeline406/1(q) -> Concat19/2
  pipeline418/1(q) -> bus_mult/2(b)
  pipeline443/1(q) -> bus_addsub/1(a)
  pipeline444/1(q) -> bus_addsub/2(b)
  wng_corr/1(bus_out) -> pipeline444/1(d)
  pipeline458/1(q) -> bus_addsub2/2(b)
  pipeline461/1(q) -> [cwg_80_1], [cwg_80_0]
  Delay46/1 -> bus_addsub4/2(b)
  Delay38/1 -> Logical46/1, Logical44/1
  Delay39/1 -> Logical45/2
  Delay40/1 -> Delay44/1
  Delay41/1 -> Delay45/1
  Delay42/1 -> Logical43/1
  Delay44/1 -> Delay47/1
  Delay45/1 -> Delay48/1
  Delay47/1 -> sample_masking/3(first_samples)
  Delay48/1 -> sample_masking/4(last_samples)
  Delay54/1 -> Logical35/2
  Delay55/1 -> Logical4/1
  Delay56/1 -> Delay57/1
  Delay57/1 -> Delay58/1
  Delay58/1 -> Delay59/1
  Delay59/1 -> sample_masking/1(timei)
  sample_masking/4(flag_valid) -> Delay60/1
  Delay60/1 -> [flag_en]
  Logical4/1 -> sample_masking/7(flag_en)  "flag_en"
  sample_masking/1(timeo) -> Delay61/1
  Delay61/1 -> [masked_time]
  [local_time] -> Delay63/1
  [en_armed] -> Delay64/1
  [local_time] -> Delay65/1, Delay67/1, Delay71/1, Delay74/1
  [start_time] -> Delay66/1
  [end_time] -> Delay68/1, Delay69/1
  Delay63/1 -> Delay56/1
  Delay64/1 -> Delay38/1
  Delay65/1 -> Relational9/1
  Delay66/1 -> Relational9/2
  Delay67/1 -> Relational17/1
  Delay68/1 -> Relational17/2
  Delay69/1 -> Relational18/1
  Delay70/1 -> Relational18/2
  Delay71/1 -> Relational19/1
  Delay72/1 -> Relational19/2
  Delay74/1 -> Relational20/1
  Delay75/1 -> Relational20/2
  Delay78/1 -> Logical42/1, Logical24/1
  Delay79/1 -> Relational4/1
  Delay80/1 -> Relational4/2
  Delay81/1 -> Relational5/1
  Delay82/1 -> Relational5/2
  Delay86/1 -> Relational8/1
  bus_convert/1(dout) -> [cwg0_tp2], pipeline461/1(d)
  Pulse Generator1/1 -> orig_control/7(sim_7)
  bus_convert2/1(dout) -> [wng0_sum], Delay139/1
  bus_convert4/1(dout) -> Delay46/1
  bus_convert6/1(dout) -> pipeline417/1(d)
  scale_out0/1(in_scale) -> Gateway Out73/1, pipeline418/1(d)
  pipeline217/1(q) -> Slice37/1
  Slice37/1 -> Convert1/1
  Convert1/1 -> [pol0_always_on]
  pipeline222/1(q) -> Slice40/1
  Slice40/1 -> Convert3/1
  [pol0_always_on] -> gbe0_traffic_control/1(always_on)
  [pol0_requested_pkts] -> gbe0_traffic_control/2(requested_pkts)
  [pol0_offset_data] -> gbe0_traffic_control/3(offset_data)
  [mrst] -> gbe0_traffic_control/4(mrst)
  [pol0_traffic_trigger] -> gbe0_traffic_control/5(traffic_trigger)
  gbe0_traffic_control/1(gbe_txen_gate) -> [gbe_txen_gate0]
  Constant174/1 -> pol1_sample_offset/1(sim_1)
  pipeline219/1(q) -> [pol1_offset_data]
  Constant173/1 -> pol0_sample_offset/1(sim_1)
  pipeline218/1(q) -> [pol0_offset_data]
  Constant175/1 -> pol0_num_pkts/1(sim_1)
  pipeline216/1(q) -> [pol0_requested_pkts]
  Constant180/1 -> pol1_num_pkts/1(sim_1)
  pipeline225/1(q) -> [pol1_requested_pkts]
  pipeline227/1(q) -> Slice38/1
  Slice38/1 -> Convert2/1
  Convert2/1 -> [pol1_always_on]
  pipeline416/1(q) -> Terminator64/1
  Delay32/1 -> pol_traffic_trigger/1(sim_1)
  Constant172/1 -> pol_tx_always_on/1(sim_1)
  Constant184/1 -> pol_tx_always_on/2(sim_2)
  pol0_num_pkts/1(in_pol0_num_pkts) -> pipeline216/1(d)
  pol1_num_pkts/1(in_pol1_num_pkts) -> pipeline225/1(d)
  pol_tx_always_on/1(in_pol0_tx_always_on) -> pipeline217/1(d)
  pol_tx_always_on/2(in_pol1_tx_always_on) -> pipeline227/1(d)
  pol0_sample_offset/1(in_pol0_sample_offset) -> pipeline218/1(d)
  pol1_sample_offset/1(in_pol1_sample_offset) -> pipeline219/1(d)
  Delay87/1 -> pol_traffic_trigger/2(sim_2)
  pol_traffic_trigger/1(in_pol0_tx_trigger) -> pipeline222/1(d)
  pipeline221/1(q) -> Slice41/1
  Slice41/1 -> Convert4/1
  Convert4/1 -> [pol1_traffic_trigger]
  pol_traffic_trigger/2(in_pol1_tx_trigger) -> pipeline221/1(d)
  edge_detect31/1(out) -> Terminator66/1  "mrst"
  Constant170/1 -> freq_cwg0/1(sim_1)
  freq_cwg0/1(in_frequency) -> pipeline411/1(d)
  AddSub2/1 -> Slice21/1
  AddSub1/1 -> Slice22/1
  [tvg_stime] -> AddSub2/1, AddSub1/1
  Constant189/1 -> speadtime0_offset/1(sim_1)
  Slice21/1 -> Register5/1
  Slice22/1 -> Register6/1
  speadtime0_offset/1(in_speadtime_offset0) -> AddSub2/2
  Constant190/1 -> speadtime1_offset/1(sim_1)
  speadtime1_offset/1(in_speadtime_offset1) -> AddSub1/2
  Convert3/1 -> [pol0_traffic_trigger]
  Constant125/1 -> scale_cwg0/2(sim_2)
  Constant179/1 -> scale_cwg0/1(sim_1)
  Constant162/1 -> scale_out0/1(sim_1)
  Constant167/1 -> scale_out0/2(sim_2)
  scale_out0/2(in_dummy) -> Terminator15/1
  gbe1_traffic_control/1(gbe_txen_gate) -> [gbe_txen_gate1]
  gbe2_traffic_control/1(gbe_txen_gate) -> [gbe_txen_gate2]
  gbe3_traffic_control/1(gbe_txen_gate) -> [gbe_txen_gate3]
  [spead_valid0] -> gbe0_traffic_control/6(spead_valid)
  [pol0_always_on] -> gbe1_traffic_control/1(always_on)
  [pol0_requested_pkts] -> gbe1_traffic_control/2(requested_pkts)
  [pol0_offset_data] -> gbe1_traffic_control/3(offset_data)
  [mrst] -> gbe1_traffic_control/4(mrst)
  [pol0_traffic_trigger] -> gbe1_traffic_control/5(traffic_trigger)
  [pol1_always_on] -> gbe2_traffic_control/1(always_on)
  [pol1_requested_pkts] -> gbe2_traffic_control/2(requested_pkts)
  [pol1_offset_data] -> gbe2_traffic_control/3(offset_data)
  [mrst] -> gbe2_traffic_control/4(mrst)
  [pol1_traffic_trigger] -> gbe2_traffic_control/5(traffic_trigger)
  [pol1_always_on] -> gbe3_traffic_control/1(always_on)
  [pol1_requested_pkts] -> gbe3_traffic_control/2(requested_pkts)
  [pol1_offset_data] -> gbe3_traffic_control/3(offset_data)
  [mrst] -> gbe3_traffic_control/4(mrst)
  [pol1_traffic_trigger] -> gbe3_traffic_control/5(traffic_trigger)
  [spead_valid1] -> gbe1_traffic_control/6(spead_valid)
  [spead_valid2] -> gbe2_traffic_control/6(spead_valid)
  [spead_valid3] -> gbe3_traffic_control/6(spead_valid)
  Constant164/1 -> Delay32/1
  Constant145/1 -> Delay87/1
  master_reset_sim7/1 -> dram_addr_offset/1(sim_1)
  master_reset_sim8/1 -> arb_rst/1(sim_1)
  master_reset_sim9/1 -> arb_en/1(sim_1)
  pipeline224/1(q) -> [arb_en0]
  pipeline229/1(q) -> [dram_addr_offset0]
  master_reset_sim1/1 -> dram_read_length/1(sim_1)
  master_reset_sim2/1 -> dram_rd_trigger/1(sim_1)
  pipeline243/1(q) -> [dram_rd_trig0]
  master_reset_sim3/1 -> dram_tvg/1(sim_1)
  master_reset_sim4/1 -> dram_tvg_length/1(sim_1)
  pipeline240/1(q) -> [dram_tvg_length0]
  edge_detect13/1(out) -> [arb_rst0]
  pipeline226/1(q) -> edge_detect13/1(in)
  master_reset_sim5/1 -> dram_rd_repeat/1(sim_1)
  pipeline244/1(q) -> [dram_rd_repeat0]
  pipeline238/1(q) -> Slice26/1, Slice24/1
  Slice26/1 -> Logical21/1, [tvg_sel0]
  Slice24/1 -> Logical21/2
  Logical21/1 -> [dram_tvg0]
  pipeline241/1(q) -> [dram_read_length0]
  master_reset_sim6/1 -> dram_rd_repeat_rate/1(sim_1)
  pipeline228/1(q) -> [dram_rd_repeat_delay0]
  [cwg_80_1] -> pipeline290/1(d)
  [cwg_80_0] -> pipeline287/1(d)
  pipeline251/1(q) -> [source_sel_0]
  pipeline252/1(q) -> [source_sel_1]
  Constant194/1 -> src_sel_cntrl/1(sim_1)
  Constant195/1 -> src_sel_cntrl/2(sim_2)
  src_sel_cntrl/1(in_src_sel_0) -> pipeline251/1(d)
  src_sel_cntrl/2(in_src_sel_1) -> pipeline252/1(d)
  [source_sel_0] -> pipeline285/1(d)
  [source_sel_1] -> pipeline289/1(d)
  Mux9/1 -> pipeline292/1(d)
  Mux8/1 -> pipeline293/1(d)
  master_reset_sim10/1 -> arb_rst/2(sim_2)
  master_reset_sim11/1 -> dram_rd_trigger/2(sim_2)
  master_reset_sim12/1 -> arb_en/2(sim_2)
  dram_rd_repeat_rate/1(in_dram_rd_repeat_rate) -> pipeline228/1(d)
  dram_rd_repeat/1(in_dram_rd_repeat) -> pipeline244/1(d)
  dram_tvg/1(in_arb_tvg) -> pipeline238/1(d)
  dram_tvg_length/1(in_tvg_length) -> pipeline240/1(d)
  dram_addr_offset/1(in_dram_addr_offset) -> pipeline229/1(d)
  dram_read_length/1(in_dram_read_length) -> pipeline241/1(d)
  dram_rd_trigger/1(in_arb_trig) -> pipeline243/1(d)
  dram_rd_trigger/2(in_dummy) -> Terminator70/1
  arb_en/1(in_arb_en) -> pipeline224/1(d)
  arb_en/2(in_dummy) -> Terminator68/1
  arb_rst/1(in_rst) -> pipeline226/1(d)
  arb_rst/2(in_dummy) -> Terminator69/1
  pipeline285/1(q) -> Mux9/1
  pipeline287/1(q) -> Mux9/2
  pipeline288/1(q) -> Mux9/3
  pipeline289/1(q) -> Mux8/1
  pipeline290/1(q) -> Mux8/2
  pipeline291/1(q) -> Mux8/3
  pipeline411/1(q) -> cwg0/1(freq)
  pipeline410/1(q) -> cwg0/2(scale)
  [mrst] -> pipeline276/1(d)
  Constant166/1 -> rpt_en_cwg0/2(sim_2)
  Constant168/1 -> rpt_length_cwg0/1(sim_1)
  rpt_en_cwg0/1(in_en) -> Convert25/1
  rpt_en_cwg0/2(in_dummy) -> Terminator71/1
  Constant177/1 -> rpt_en_cwg0/1(sim_1)
  Convert25/1 -> pipeline277/1(d)
  cwg0/1(bus_out) -> pipeline457/1(d), [Bus_expand_cwg0]
  rpt_length_cwg0/1(in_cwg0_repeat_length) -> pipeline278/1(d)
  pipeline276/1(q) -> cwg0/3(rst)
  pipeline277/1(q) -> cwg0/4(repeat_en)
  pipeline278/1(q) -> cwg0/5(repeat_length)
  [adc_count] -> Concat20/1
  Constant198/1 -> Concat20/2
  Delay73/1 -> [status0]
  Delay90/1 -> [status3]
  Delay89/1 -> [status2]
  Delay88/1 -> [status1]
  Concat20/1 -> Delay90/1, Delay73/1, Delay88/1, Delay89/1
  [ndiode_flag] -> Convert28/1
  Logical/1 -> Convert27/1
  Logical23/1 -> Convert30/1
  [adc_flag] -> Convert29/1
  [flag_en] -> Logical/1, Logical23/2
  Convert28/1 -> Logical/2
  Convert29/1 -> Logical23/1
  Convert30/1 -> Concat20/3
  Convert27/1 -> Concat20/4
  cwg0/3(rpt_rst) -> Terminator74/1
  pipeline295/1(q) -> wng0/2(rst)
  Constant89/1 -> man_rst_wng0/1(sim_1)
  Logical25/1 -> pipeline295/1(d)
  man_rst_wng0/1(in_rst) -> [wng0_man_rst], Logical25/2
  Gateway Out33/1 -> To Workspace33/1
  [wng0_rst] -> Logical25/1
  [local_time] -> pipeline302/1(d)
  [mrst] -> pipeline300/1(d)
  [wng0_man_rst] -> pipeline296/1(d)
  wng_rst/1(wng_rst) -> Gateway Out33/1, [wng0_rst]
  Constant196/1 -> rpt_length_wng0/1(sim_1)
  pipeline299/1(q) -> wng_rst/5(num_samples_for_rst)
  pipeline296/1(q) -> wng_rst/4(man_rst)
  pipeline300/1(q) -> wng_rst/3(mrst)
  pipeline301/1(q) -> wng_rst/2(future_time)
  pipeline302/1(q) -> wng_rst/1(local_time)
  Constant203/1 -> rpt_load_time_msw_wng0/1(sim_1)
  Constant201/1 -> rpt_load_time_lsw_wng0/1(sim_1)
  Concat17/1 -> Delay33/1
  pipeline303/1(q) -> Concat17/1
  pipeline304/1(q) -> Concat17/2
  rpt_load_time_lsw_wng0/1(in_reg) -> pipeline304/1(d)
  rpt_load_time_msw_wng0/1(in_reg) -> pipeline303/1(d)
  Delay33/1 -> pipeline301/1(d)
  rpt_length_wng0/1(in_samples) -> pipeline305/1(d)
  pipeline305/1(q) -> pipeline299/1(d)
  [local_time] -> pipeline247/1(d)
  Impulse/1(impulse0) -> [Impulse_gen0]
  pipeline245/1(q) -> Impulse/2(future_time)
  pipeline247/1(q) -> Impulse/1(local_time)
  Constant200/1 -> impulse_load_time_msw/1(sim_1)
  Constant199/1 -> impulse_load_time_lsw/1(sim_1)
  Concat21/1 -> Delay35/1
  pipeline248/1(q) -> Concat21/1
  pipeline254/1(q) -> Concat21/2
  impulse_load_time_lsw/1(in_reg) -> pipeline254/1(d)
  impulse_load_time_msw/1(in_reg) -> pipeline248/1(d)
  Delay35/1 -> pipeline245/1(d)
  pipeline257/1(q) -> Mux9/4
  [Impulse_gen0] -> pipeline257/1(d)
  pipeline258/1(q) -> Mux8/4
  [Impulse_gen0] -> pipeline258/1(d)
  gpio/1 -> Terminator75/1
  Gateway Out/1 -> To Workspace/1
  Impulse/2(impulse_gpio) -> [Impulse_gpio]
  pipeline237/1(q) -> Impulse/3(delay_correction)
  impulse_delay_correction/1(in_reg) -> pipeline237/1(d)
  Constant160/1 -> impulse_delay_correction/1(sim_1)
  pipeline236/1(q) -> Gateway Out/1, gpio/1
  [Impulse_gpio] -> pipeline236/1(d)
  pipeline417/1(q) -> [cwg0_tp0], bus_mult/1(a)
  Logical29/1 -> pipeline260/1(d)
  man_rst_wng_corr/1(in_rst) -> Logical29/2
  [wng0_rst] -> Logical29/1
  Constant101/1 -> man_rst_wng_corr/1(sim_1)
  Gateway Out73/1 -> To Workspace73/1
  Gateway Out84/1 -> To Workspace84/1
  Gateway Out37/1 -> To Workspace37/1
  Constant103/1 -> scale_wng0/2(sim_2)
  Constant104/1 -> pipeline288/1(d)
  Constant105/1 -> pipeline291/1(d)
  [tvg_ltime] -> Delay36/1
  Delay36/1 -> Delay37/1
  [data_80_0] -> Delay91/1
  Delay91/1 -> Delay92/1
  bus_expand17/7(out2) -> pipeline261/1(d)
  bus_expand17/8(lsb_out1) -> pipeline265/1(d)
  bus_expand17/6(out3) -> pipeline266/1(d)
  bus_expand17/5(out4) -> pipeline267/1(d)
  bus_expand17/4(out5) -> pipeline308/1(d)
  bus_expand17/3(out6) -> pipeline310/1(d)
  bus_expand17/2(out7) -> pipeline311/1(d)
  bus_expand17/1(msb_out8) -> pipeline312/1(d)
  pipeline312/1(q) -> ss_fifo_in/1(in_d0)
  pipeline311/1(q) -> ss_fifo_in/2(in_d1)
  pipeline310/1(q) -> ss_fifo_in/3(in_d2)
  pipeline308/1(q) -> ss_fifo_in/4(in_d3)
  pipeline267/1(q) -> ss_fifo_in/5(in_d4)
  pipeline266/1(q) -> ss_fifo_in/6(in_d5)
  pipeline261/1(q) -> ss_fifo_in/7(in_d6)
  pipeline265/1(q) -> ss_fifo_in/8(in_d7)
  Delay92/1 -> bus_expand17/1(bus_in)
  Delay37/1 -> pipeline315/1(d), Relational22/1
  pipeline315/1(q) -> ss_localtime/1(in_time)
  pipeline313/1(q) -> ss_fifo_in/9(in_gpio_trig)
  Delay93/1 -> Delay94/1
  Delay94/1 -> pipeline313/1(d)
  [Impulse_gpio] -> Delay96/1
  Delay96/1 -> Delay93/1
  pipeline314/1(q) -> Impulse/4(Impulse_offset)
  Constant109/1 -> impulse_offset/1(sim_1)
  impulse_offset/1(in_reg) -> pipeline314/1(d)
  Constant108/1 -> ss_trig_time_msw/1(sim_1)
  Constant107/1 -> ss_trig_time_lsw/1(sim_1)
  Concat23/1 -> Delay97/1
  pipeline316/1(q) -> Concat23/1
  pipeline317/1(q) -> Concat23/2
  ss_trig_time_lsw/1(in_reg) -> pipeline317/1(d)
  ss_trig_time_msw/1(in_reg) -> pipeline316/1(d)
  Delay97/1 -> Relational22/2
  Relational22/1 -> edge_detect/1
  pipeline318/1(q) -> ss_fifo_in/10(we)
  [fifoselect] -> pipeline319/1(d), pipeline318/1(d)
  pipeline319/1(q) -> ss_localtime/2(we)
  edge_detect/1 -> ss_fifo_in/11(trig), ss_localtime/3(trig)
  Constant111/1 -> start_load_time_msw/1(sim_1)
  Constant110/1 -> start_load_time_lsw/1(sim_1)
  pipeline321/1(q) -> Concat24/1
  pipeline322/1(q) -> Concat24/2
  start_load_time_msw/1(in_reg) -> pipeline321/1(d)
  start_load_time_lsw/1(in_reg) -> pipeline322/1(d)
  Concat24/1 -> Delay98/1
  Constant113/1 -> stop_load_time_msw/1(sim_1)
  Constant112/1 -> stop_load_time_lsw/1(sim_1)
  pipeline323/1(q) -> Concat12/1
  pipeline324/1(q) -> Concat12/2
  stop_load_time_msw/1(in_reg) -> pipeline323/1(d)
  stop_load_time_lsw/1(in_reg) -> pipeline324/1(d)
  Concat12/1 -> Delay99/1
  Delay98/1 -> pipeline326/1(d)
  Delay99/1 -> pipeline325/1(d)
  pipeline326/1(q) -> Start_stop_Cntrl/1(start_time)
  pipeline325/1(q) -> Start_stop_Cntrl/2(stop_time)
  [mrst] -> Start_stop_Cntrl/3(rst)
  Start_stop_Cntrl/1(Start_Stop_Sel) -> [Start_Stop_Sel]
  pipeline292/1(q) -> Mux7/2
  Mux7/1 -> [data_80_0]
  [Start_Stop_Sel] -> Mux7/1
  Mux24/1 -> [data_80_1]
  pipeline293/1(q) -> Mux24/2
  Constant114/1 -> Mux24/3
  [Start_Stop_Sel] -> Mux24/1
  Constant115/1 -> Mux7/3
  Constant106/1 -> cwg0/6(en)
  pipeline457/1(q) -> bus_addsub2/1(a)
  edge_detect16/1(out) -> pipeline263/1(d)
  control1/4(in_cnt_rst) -> edge_detect14/1(in)
  edge_detect14/1(out) -> pipeline235/1(d)
  control1/3(in_gbe_rst) -> pipeline268/1(d)
  control1/1(in_sys_rst) -> pipeline246/1(d)
  pipeline246/1(q) -> [sys_rst]
  pipeline263/1(q) -> [clr_status]
  pipeline268/1(q) -> [gbe_rst]
  pipeline235/1(q) -> [cnt_rst]
  edge_detect15/1(out) -> pipeline249/1(d)
  pipeline249/1(q) -> [gbe_cnt_rst]
  control1/5(in_gbe_cnt_rst) -> edge_detect15/1(in)
  control1/2(in_status_clr) -> edge_detect16/1(in)
  [forty_gbe_led_up] -> Delay114/1
  [forty_gbe_led_rx] -> Delay101/1
  [forty_gbe_led_tx] -> Delay110/1
  [forty_gbe_tx_afull] -> Delay107/1
  [forty_gbe_tx_overflow] -> Delay112/1
  [forty_gbe_rx_overrun] -> Delay111/1
  [arb_rst0] -> Terminator84/1
  [arb_en0] -> Terminator26/1
  [dram_rd_repeat0] -> Terminator27/1
  [dram_rd_repeat_delay0] -> Terminator29/1
  [tvg_sel0] -> Terminator30/1
  [dram_tvg0] -> Terminator33/1
  [dram_tvg_length0] -> Terminator34/1
  [dram_addr_offset0] -> Terminator36/1
  [dram_read_length0] -> Terminator37/1
  cwg0/2(dvalid) -> Terminator42/1
  Delay107/1 -> status0/4(out_tx_afull)
  Delay101/1 -> status0/2(out_led_rx)
  Delay112/1 -> status0/5(out_tx_overflow)
  Delay111/1 -> status0/6(out_rx_overrun)
  Delay110/1 -> status0/3(out_led_tx)
  Delay114/1 -> status0/1(out_led_up)
  pipeline242/1(q) -> [gbe_port]
  scale_wng0/1(in_scale) -> Gateway Out37/1, pipeline407/1(d)
  pipeline408/1(q) -> wng_corr/1(scale_16_14)
  pipeline260/1(q) -> wng_corr/2(rst)
  Constant193/1 -> scale_wng_corr/2(sim_2)
  Gateway Out32/1 -> To Workspace95/1
  scale_wng_corr/1(in_scale) -> Gateway Out32/1, pipeline408/1(d)
  [cwg_80_0] -> Delay120/1
  Delay120/1 -> Delay121/1
  bus_expand5/7(out2) -> pipeline456/1(d)
  bus_expand5/8(lsb_out1) -> pipeline231/1(d)
  bus_expand5/6(out3) -> pipeline253/1(d)
  bus_expand5/5(out4) -> pipeline214/1(d)
  bus_expand5/4(out5) -> pipeline215/1(d)
  bus_expand5/3(out6) -> pipeline230/1(d)
  bus_expand5/2(out7) -> pipeline232/1(d)
  bus_expand5/1(msb_out8) -> pipeline233/1(d)
  pipeline233/1(q) -> ss_cwg0/1(in_d0)
  pipeline232/1(q) -> ss_cwg0/2(in_d1)
  pipeline230/1(q) -> ss_cwg0/3(in_d2)
  pipeline215/1(q) -> ss_cwg0/4(in_d3)
  pipeline214/1(q) -> ss_cwg0/5(in_d4)
  pipeline253/1(q) -> ss_cwg0/6(in_d5)
  pipeline456/1(q) -> ss_cwg0/7(in_d6)
  pipeline231/1(q) -> ss_cwg0/8(in_d7)
  Delay121/1 -> bus_expand5/1(bus_in)
  pipeline234/1(q) -> ss_cwg0/9(in_gpio_trig)
  pipeline250/1(q) -> edge_detect29/1, ss_cwg0/10(we)
  Delay122/1 -> Delay123/1
  [Impulse_gpio] -> Delay122/1
  Delay123/1 -> pipeline234/1(d)
  [fifoselect] -> pipeline250/1(d)
  edge_detect29/1 -> ss_cwg0/11(trig)
  scale_cwg0/1(in_scale) -> Gateway Out36/1, pipeline410/1(d)
  Gateway Out36/1 -> To Workspace228/1
  [gbe_rst] -> forty_gbe/1(rst)
  Constant83/1 -> forty_gbe/7(rx_ack)
  Constant161/1 -> forty_gbe/8(rx_overrun_ack)
  [clr_status] -> forty_gbe/9(debug_rst)
  [sp256_eof] -> forty_gbe/6(tx_end_of_frame)
  [sp256_dv4] -> forty_gbe/3(tx_valid)
  [sp256_data] -> forty_gbe/2(tx_data)
  [gbe_port] -> forty_gbe/5(tx_dest_port)
  [gbe_txip] -> forty_gbe/4(tx_dest_ip)
  pipeline359/1(q) -> [forty_gbe_led_up]
  pipeline362/1(q) -> [forty_gbe_led_rx]
  pipeline357/1(q) -> [forty_gbe_led_tx]
  pipeline358/1(q) -> [forty_gbe_tx_afull]
  pipeline360/1(q) -> [forty_gbe_tx_overflow]
  forty_gbe/1(led_up) -> pipeline359/1(d)
  forty_gbe/2(led_rx) -> pipeline362/1(d)
  forty_gbe/3(led_tx) -> pipeline357/1(d)
  forty_gbe/4(tx_afull) -> pipeline358/1(d)
  forty_gbe/5(tx_overflow) -> pipeline360/1(d)
  pipeline363/1(q) -> [forty_gbe_rx_overrun]
  forty_gbe/12(rx_overrun) -> pipeline363/1(d)
  forty_gbe/14(rx_dest_port) -> Terminator45/1
  forty_gbe/13(rx_dest_ip) -> Terminator46/1
  forty_gbe/11(rx_bad_frame) -> Terminator47/1
  forty_gbe/10(rx_end_of_frame) -> Terminator48/1
  forty_gbe/9(rx_source_port) -> Terminator49/1
  forty_gbe/8(rx_source_ip) -> Terminator50/1
  forty_gbe/7(rx_valid) -> Terminator51/1
  forty_gbe/6(rx_data) -> Terminator52/1
  gbecontrol/1(in_gbe0) -> [gbe_txen0]
  gbecontrol/2(in_gbe1) -> [gbe_txen1]
  gbecontrol/3(in_gbe2) -> [gbe_txen2]
  gbecontrol/4(in_gbe3) -> [gbe_txen3]
  ramp0/1 -> [rampdata0]
  [vld0] -> ramp0/2
  [rdy0] -> ramp0/1
  ramp1/1 -> [rampdata1]
  [vld1] -> ramp1/2
  [rdy1] -> ramp1/1
  speadsnap_control/1(in_speadsnap_arm) -> Delay100/1
  Delay100/1 -> [speadsnap_arm]
  ramp2/1 -> [rampdata2]
  [vld2] -> ramp2/2
  [rdy2] -> ramp2/1
  ramp3/1 -> [rampdata3]
  [vld3] -> ramp3/2
  [rdy3] -> ramp3/1
  Constant116/1 -> gbecontrol/2(sim_2)
  Constant202/1 -> gbecontrol/1(sim_1)
  Constant117/1 -> gbecontrol/3(sim_3)
  Constant118/1 -> gbecontrol/4(sim_4)
  ramp80/1 -> [ramp79]
  [rst_ramp80] -> ramp80/1
  Delay102/1 -> [sel_ramp80]
  test_control/1(in_sel_ramp80) -> Delay102/1
  Delay103/1 -> [rst_ramp80]
  test_control/2(in_rst_ramp80) -> Delay103/1
  fifo4/1(fifo_data80) -> pipeline389/1(d)  "data00"
  fifo4/2(fifo_dv) -> Gateway Out82/1, pipeline390/1(d)  "dv00"
  fifo4/3(word_start) -> Gateway Out83/1, pipeline391/1(d)  "ws00"
  fifo4/4(pkt_start) -> Gateway Out85/1, pipeline392/1(d)  "ps00"
  fifo4/5(fifo_full) -> Terminator40/1  "full00"
  fifo4/6(fifo_empty) -> Terminator56/1  "empty00"
  fifo5/1(fifo_data80) -> pipeline430/1(d)  "data01"
  fifo5/2(fifo_dv) -> Gateway Out79/1, pipeline431/1(d)  "dv01"
  fifo5/3(word_start) -> Gateway Out80/1, pipeline432/1(d)  "ws01"
  fifo5/4(pkt_start) -> Gateway Out81/1, pipeline433/1(d)  "ps01"
  pack_80_64_5/2(valid64) -> pipeline449/1(d)  "v64_01"
  pack_80_64_5/1(ready64) -> pipeline448/1(d)  "r64_01"
  fifo5/5(fifo_full) -> Terminator41/1
  fifo5/6(fifo_empty) -> Terminator54/1
  [hdr_0x3101] -> bus_create10/1(in1)
  [pol0_id] -> bus_create10/2(in2)
  [hdr_0x3101] -> bus_create4/1(in1)
  [pol0_id] -> bus_create4/2(in2)
  [speadtime0] -> spead_pack4/8(hdr5_0x1600_DIR), spead_pack4/4(hdr_heap_id)  "timein0"
  bus_create10/1(bus_out) -> spead_pack4/9(hdr6_0x3101_DIR)
  [status0] -> spead_pack4/10(hdr7_0x3102_DIR)
  bus_create4/1(bus_out) -> spead_pack5/9(hdr6_0x3101_DIR)
  [status1] -> spead_pack5/10(hdr7_0x3102_DIR)
  [tvg_ltime] -> fifo_select1/1(localtime)
  fifo_select1/1(fifo_select0) -> fifo4/2(fifo_we_en), Gateway Out52/1, [fifoselect]  "fifoselect"
  [speadtime1] -> spead_pack5/4(hdr_heap_id), spead_pack5/8(hdr5_0x1600_DIR)  "timein1"
  pack_80_64_4/1(ready64) -> pipeline446/1(d)  "r64_00"
  pack_80_64_4/2(valid64) -> pipeline447/1(d)  "v64_00"
  [spead_heapsize] -> spead_pack4/5(hdr_heap_size)
  [spead_heapoffset] -> spead_pack4/6(hdr_heap_offset)
  [spead_pktlen] -> spead_pack4/7(hdr_pkt_len_words)
  [spead_heapsize] -> spead_pack5/5(hdr_heap_size)
  [spead_heapoffset] -> spead_pack5/6(hdr_heap_offset)
  [spead_pktlen] -> spead_pack5/7(hdr_pkt_len_words)
  spead_pack5/4(data_overflow) -> Terminator39/1
  [adc_data_offset] -> spead_pack4/11(hdr8_0x3300)
  [adc_data_offset] -> spead_pack5/11(hdr8_0x3300)
  Constant121/1 -> [spead_heapsize]
  Constant122/1 -> [spead_pktlen]
  Constant126/1 -> [spead_heapoffset]
  spead_pack4/4(data_overflow) -> Terminator38/1
  spead_pack4/3(eof) -> pipeline334/1(d)
  spead_pack4/1(data_out) -> pipeline330/1(d)  "packd"
  spead_pack4/2(valid_out) -> pipeline333/1(d)  "packv"
  spead_pack5/1(data_out) -> pipeline340/1(d)
  spead_pack5/2(valid_out) -> pipeline341/1(d)
  spead_pack5/3(eof) -> pipeline342/1(d)
  Constant141/1 -> [adc_data_offset]
  pipeline330/1(q) -> Gateway Out129/1, [spead_data0]
  pipeline333/1(q) -> [spead_valid0]  "sp_dv0"
  pipeline334/1(q) -> [spead_eof0]
  pipeline340/1(q) -> [spead_data1]
  pipeline341/1(q) -> [spead_valid1]  "sp_dv1"
  pipeline342/1(q) -> [spead_eof1]
  pipeline389/1(q) -> Mux12/2  "d80"
  pipeline390/1(q) -> pack_80_64_4/2(valid80)  "v80"
  pipeline391/1(q) -> pack_80_64_4/3(word_start)  "wd_start"
  pipeline392/1(q) -> Delay109/1, pack_80_64_4/4(pkt_start)  "pkt_start"
  pipeline430/1(q) -> Mux13/2
  pipeline431/1(q) -> pack_80_64_5/2(valid80)
  pipeline432/1(q) -> pack_80_64_5/3(word_start)
  pipeline433/1(q) -> Delay113/1, pack_80_64_5/4(pkt_start)
  pipeline446/1(q) -> [rdy0], spead_pack4/1(data64_ready)
  pipeline447/1(q) -> [vld0], spead_pack4/2(data64_valid)
  pipeline448/1(q) -> [rdy1], spead_pack5/1(data64_ready)
  pipeline449/1(q) -> [vld1], spead_pack5/2(data64_valid)
  fifo_select1/2(fifo_select1) -> Gateway Out59/1, fifo5/2(fifo_we_en)
  Mux20/1 -> spead_pack4/3(data64)
  Mux21/1 -> spead_pack5/3(data64)
  [spead_data0] -> pipeline451/1(d)
  [spead_valid0] -> pipeline452/1(d)
  wr_addr0/1 -> Gateway Out57/1, 64_to_256/1  "waddr"
  [spead_valid0] -> edge_detect28/1(in), edge_detect39/1, pipeline450/1(d)
  Constant129/1 -> 64_to_256/6
  Constant130/1 -> 64_to_256/5
  rd_addr0/1 -> Gateway Out56/1, 64_to_256/4, Relational23/2  "rdaddr"
  64_to_256/2 -> pipeline270/1(d)
  edge_detect39/1 -> wr_addr0/1
  pipeline450/1(q) -> wr_addr0/2
  pipeline451/1(q) -> 64_to_256/2
  pipeline452/1(q) -> 64_to_256/3  "dv64_0"
  64_to_256/1 -> Terminator61/1
  edge_detect28/1(out) -> rd_addr0/1, rd_arm/3, Gateway Out55/1, rd_arm/1
  Constant140/1 -> Relational23/1
  Relational23/1 -> Gateway Out54/1, rd_arm/2  "rd_done"
  rd_arm/1 -> Gateway Out53/1, pipeline453/1(d), Gateway Out58/1, 64_to_256/7, rd_addr0/2  "rd_en"
  pipeline453/1(q) -> edge_detect8/1(in), pipeline223/1(d)
  edge_detect8/1(out) -> Gateway Out48/1, [sp256_eof0]  "eof256_0"
  fifo6/1(fifo_data80) -> pipeline348/1(d)  "data00"
  fifo6/2(fifo_dv) -> Gateway Out72/1, pipeline349/1(d)  "dv00"
  fifo6/3(word_start) -> Gateway Out74/1, pipeline351/1(d)  "ws00"
  fifo6/4(pkt_start) -> Gateway Out75/1, pipeline352/1(d)  "ps00"
  fifo6/5(fifo_full) -> Terminator57/1  "full00"
  fifo6/6(fifo_empty) -> Terminator60/1  "empty00"
  fifo7/1(fifo_data80) -> pipeline271/1(d)  "data01"
  fifo7/2(fifo_dv) -> Gateway Out76/1, pipeline272/1(d)  "dv01"
  fifo7/3(word_start) -> Gateway Out77/1, pipeline273/1(d)  "ws01"
  fifo7/4(pkt_start) -> Gateway Out78/1, pipeline274/1(d)  "ps01"
  pack_80_64_7/2(valid64) -> pipeline328/1(d)  "v64_01"
  pack_80_64_7/1(ready64) -> pipeline327/1(d)  "r64_01"
  fifo7/5(fifo_full) -> Terminator58/1
  fifo7/6(fifo_empty) -> Terminator59/1
  [hdr_0x3101] -> bus_create6/1(in1)
  [pol1_id] -> bus_create6/2(in2)
  [hdr_0x3101] -> bus_create5/1(in1)
  [pol1_id] -> bus_create5/2(in2)
  [speadtime0] -> spead_pack6/4(hdr_heap_id), spead_pack6/8(hdr5_0x1600_DIR)  "timein0"
  bus_create6/1(bus_out) -> spead_pack6/9(hdr6_0x3101_DIR)
  [status2] -> spead_pack6/10(hdr7_0x3102_DIR)
  bus_create5/1(bus_out) -> spead_pack7/9(hdr6_0x3101_DIR)
  [status3] -> spead_pack7/10(hdr7_0x3102_DIR)
  fifo_select2/1(fifo_select0) -> Gateway Out71/1, fifo6/2(fifo_we_en)  "fifoselect"
  [speadtime1] -> spead_pack7/8(hdr5_0x1600_DIR), spead_pack7/4(hdr_heap_id)  "timein1"
  pack_80_64_6/1(ready64) -> pipeline294/1(d)  "r64_00"
  pack_80_64_6/2(valid64) -> pipeline307/1(d)  "v64_00"
  [spead_heapsize] -> spead_pack6/5(hdr_heap_size)
  [spead_heapoffset] -> spead_pack6/6(hdr_heap_offset)
  [spead_pktlen] -> spead_pack6/7(hdr_pkt_len_words)
  [spead_heapsize] -> spead_pack7/5(hdr_heap_size)
  [spead_heapoffset] -> spead_pack7/6(hdr_heap_offset)
  [spead_pktlen] -> spead_pack7/7(hdr_pkt_len_words)
  Assert3/1 -> fifo6/1(data80), fifo7/1(data80)
  spead_pack7/4(data_overflow) -> Terminator53/1
  [adc_data_offset] -> spead_pack6/11(hdr8_0x3300)
  [adc_data_offset] -> spead_pack7/11(hdr8_0x3300)
  spead_pack6/4(data_overflow) -> Terminator79/1
  spead_pack6/3(eof) -> pipeline344/1(d)
  spead_pack6/1(data_out) -> pipeline329/1(d)  "packd"
  spead_pack6/2(valid_out) -> pipeline343/1(d)  "packv"
  spead_pack7/1(data_out) -> pipeline345/1(d)
  spead_pack7/2(valid_out) -> pipeline346/1(d)
  spead_pack7/3(eof) -> pipeline347/1(d)
  pipeline329/1(q) -> [spead_data2]
  pipeline343/1(q) -> [spead_valid2]  "sp_dv0"
  pipeline344/1(q) -> [spead_eof2]
  pipeline345/1(q) -> [spead_data3]
  pipeline346/1(q) -> [spead_valid3]  "sp_dv1"
  pipeline347/1(q) -> [spead_eof3]
  pipeline349/1(q) -> pack_80_64_6/2(valid80)
  pipeline351/1(q) -> pack_80_64_6/3(word_start)
  pipeline352/1(q) -> Delay117/1, pack_80_64_6/4(pkt_start)
  pipeline272/1(q) -> pack_80_64_7/2(valid80)
  pipeline273/1(q) -> pack_80_64_7/3(word_start)
  pipeline274/1(q) -> Delay104/1, pack_80_64_7/4(pkt_start)
  pipeline294/1(q) -> spead_pack6/1(data64_ready), [rdy2]
  pipeline307/1(q) -> spead_pack6/2(data64_valid), [vld2]
  pipeline327/1(q) -> spead_pack7/1(data64_ready), [rdy3]
  pipeline328/1(q) -> spead_pack7/2(data64_valid), [vld3]
  fifo_select2/2(fifo_select1) -> Gateway Out70/1, fifo7/2(fifo_we_en)
  Mux11/1 -> spead_pack7/3(data64)
  [spead_data2] -> pipeline354/1(d)
  [spead_valid2] -> pipeline355/1(d)
  wr_addr2/1 -> 64_to_1/1  "waddr"
  [spead_valid2] -> pipeline353/1(d), edge_detect18/1, edge_detect21/1(in)
  Constant119/1 -> 64_to_1/6
  Constant120/1 -> 64_to_1/5
  rd_addr2/1 -> Relational13/2, 64_to_1/4  "rdaddr"
  64_to_1/2 -> pipeline365/1(d)
  edge_detect18/1 -> wr_addr2/1
  pipeline353/1(q) -> wr_addr2/2
  pipeline354/1(q) -> 64_to_1/2
  pipeline355/1(q) -> 64_to_1/3  "dv64_2"
  64_to_1/1 -> Terminator62/1
  edge_detect21/1(out) -> rd_addr2/1
  Constant128/1 -> Relational13/1
  Relational13/1 -> rd_arm2/2  "rd_done"
  rd_arm2/1 -> 64_to_1/7, rd_addr2/2, pipeline356/1(d)  "rd_en"
  pipeline356/1(q) -> edge_detect19/1(in), pipeline364/1(d)  "dv256"
  edge_detect19/1(out) -> Gateway Out91/1, [sp256_eof2]  "eof256_2"
  pipeline364/1(q) -> Gateway Out90/1, [sp256_dv2]  "dv256_2"
  pipeline365/1(q) -> [sp256_data2]
  [sp256_eof0] -> rd_arm2/3, rd_arm2/1
  [spead_data1] -> pipeline367/1(d)
  [spead_valid1] -> pipeline368/1(d)
  wr_addr1/1 -> 64_to_2/1  "waddr"
  [spead_valid1] -> pipeline366/1(d), edge_detect22/1, edge_detect24/1(in)
  Constant131/1 -> 64_to_2/6
  Constant132/1 -> 64_to_2/5
  rd_addr1/1 -> Relational6/2, 64_to_2/4  "rdaddr"
  64_to_2/2 -> pipeline371/1(d)
  edge_detect22/1 -> wr_addr1/1
  pipeline366/1(q) -> wr_addr1/2
  pipeline367/1(q) -> 64_to_2/2
  pipeline368/1(q) -> 64_to_2/3  "dv64_1"
  64_to_2/1 -> Terminator63/1
  edge_detect24/1(out) -> rd_arm1/3, rd_arm1/1, rd_addr1/1
  Constant133/1 -> Relational6/1
  Relational6/1 -> rd_arm1/2  "rd_done"
  rd_arm1/1 -> 64_to_2/7, rd_addr1/2, pipeline369/1(d)  "rd_en"
  pipeline369/1(q) -> pipeline370/1(d), edge_detect23/1(in)  "dv256"
  edge_detect23/1(out) -> Gateway Out89/1, [sp256_eof1]  "eof256_1"
  pipeline370/1(q) -> Gateway Out88/1, [sp256_dv1]  "dv256_1"
  pipeline371/1(q) -> [sp256_data1]
  [spead_data3] -> pipeline374/1(d)
  [spead_valid3] -> pipeline375/1(d)
  wr_addr3/1 -> 64_to_3/1  "waddr"
  [spead_valid3] -> edge_detect27/1(in), edge_detect25/1, pipeline373/1(d)
  Constant134/1 -> 64_to_3/6
  Constant135/1 -> 64_to_3/5
  rd_addr3/1 -> 64_to_3/4, Relational11/2  "rdaddr"
  64_to_3/2 -> pipeline378/1(d)
  edge_detect25/1 -> wr_addr3/1
  pipeline373/1(q) -> wr_addr3/2
  pipeline374/1(q) -> 64_to_3/2
  pipeline375/1(q) -> 64_to_3/3  "dv64_3"
  64_to_3/1 -> Terminator81/1
  edge_detect27/1(out) -> rd_addr3/1
  Constant136/1 -> Relational11/1
  Relational11/1 -> rd_arm3/2  "rd_done"
  rd_arm3/1 -> pipeline376/1(d), 64_to_3/7, rd_addr3/2  "rd_en"
  pipeline376/1(q) -> edge_detect26/1(in), pipeline377/1(d)  "dv256"
  edge_detect26/1(out) -> Gateway Out93/1, [sp256_eof3]  "eof256_3"
  pipeline377/1(q) -> Gateway Out92/1, [sp256_dv3]  "dv256_3"
  pipeline378/1(q) -> [sp256_data3]
  [sp256_eof1] -> rd_arm3/1, rd_arm3/3
  [sp256_dv0] -> Mux6/1
  [sp256_data0] -> Mux6/3
  [sp256_data2] -> Mux6/2
  [sp256_dv1] -> pipeline436/1(d)
  Mux6/1 -> Mux25/2
  [sp256_data1] -> pipeline379/1(d)
  [sp256_dv3] -> pipeline437/1(d)
  Mux25/1 -> Mux26/2
  [sp256_data3] -> pipeline380/1(d)
  Mux26/1 -> munge/1(din)
  pipeline379/1(q) -> Mux25/3
  pipeline380/1(q) -> pipeline381/1(d)
  pipeline381/1(q) -> Mux26/3
  [sp256_dvg0] -> Gateway Out35/1, Logical39/1
  [sp256_dvg1] -> Gateway Out39/1, Logical39/2
  [sp256_dvg2] -> Gateway Out41/1, Logical39/3
  [sp256_dvg3] -> Gateway Out42/1, Logical39/4
  Logical39/1 -> pipeline386/1(d)
  pipeline386/1(q) -> pipeline387/1(d)
  pipeline387/1(q) -> Gateway Out40/1, [sp256_dv]
  [sp256_eofg0] -> Gateway Out239/1, Logical8/1
  [sp256_eofg1] -> Gateway Out30/1, Logical8/2
  [sp256_eofg2] -> Gateway Out31/1, Logical8/3
  [sp256_eofg3] -> Gateway Out34/1, Logical8/4
  Logical8/1 -> pipeline388/1(d)
  pipeline388/1(q) -> pipeline435/1(d)
  pipeline435/1(q) -> Gateway Out62/1, [sp256_eof]  "tx_eof"
  [sp256_eof] -> Mux16/1
  Constant139/1 -> Mux16/3
  Constant138/1 -> Mux16/2
  Mux16/1 -> Mux27/3
  Constant137/1 -> Mux27/2
  [sp256_dv] -> Gateway Out29/1, [sp256_dv4], Mux27/1
  [sp256_dv0] -> Mux17/1
  [gbe_ip2] -> Gateway Out45/1, Mux17/2
  [sp256_dv1] -> pipeline421/1(d)
  Mux17/1 -> Mux18/2
  [gbe_ip1] -> Gateway Out44/1, pipeline382/1(d)
  [sp256_dv3] -> pipeline422/1(d)
  Mux18/1 -> Mux19/2
  [gbe_ip3] -> Gateway Out46/1, pipeline384/1(d)
  Mux19/1 -> [gbe_txip]
  pipeline382/1(q) -> Mux18/3
  pipeline384/1(q) -> pipeline385/1(d)
  pipeline385/1(q) -> Mux19/3
  [gbe_txen0] -> Logical9/2
  pipeline223/1(q) -> Gateway Out49/1, [sp256_dv0]  "dv256_0"
  [sp256_eof0] -> Logical9/1
  [sp256_dv0] -> Logical13/1
  [gbe_txen0] -> Logical13/2
  Logical13/1 -> [sp256_dvg0]
  Logical9/1 -> [sp256_eofg0]
  [gbe_txen1] -> Logical17/2
  [sp256_eof1] -> Logical17/1
  [sp256_dv1] -> Logical18/1
  [gbe_txen1] -> Logical18/2
  Logical18/1 -> [sp256_dvg1]
  Logical17/1 -> [sp256_eofg1]
  [gbe_txen2] -> Logical19/2
  [sp256_eof2] -> Logical19/1
  [sp256_dv2] -> Logical20/1
  [gbe_txen2] -> Logical20/2
  Logical20/1 -> [sp256_dvg2]
  Logical19/1 -> [sp256_eofg2]
  [gbe_txen3] -> Logical47/2
  [sp256_eof3] -> Logical47/1
  [sp256_dv3] -> Logical22/1
  [gbe_txen3] -> Logical22/2
  Logical22/1 -> [sp256_dvg3]
  Logical47/1 -> [sp256_eofg3]
  [sp256_dvg0] -> Logical30/1
  [sp256_dvg1] -> Logical27/1
  Logical27/1 -> Logical30/2
  [sp256_dvg3] -> Logical27/3
  [sp256_dvg2] -> Logical27/2
  [sp256_dvg1] -> Logical31/1
  [sp256_dvg0] -> Logical28/1
  Logical28/1 -> Logical31/2
  [sp256_dvg3] -> Logical28/3
  [sp256_dvg2] -> Logical28/2
  [sp256_dvg2] -> Logical33/1
  [sp256_dvg0] -> Logical32/1
  Logical32/1 -> Logical33/2
  [sp256_dvg3] -> Logical32/3
  [sp256_dvg1] -> Logical32/2
  [sp256_dvg3] -> Logical36/1
  [sp256_dvg0] -> Logical34/1
  Logical34/1 -> Logical36/2
  [sp256_dvg2] -> Logical34/3
  [sp256_dvg1] -> Logical34/2
  Logical30/1 -> Logical37/1
  Logical31/1 -> Logical37/2
  Logical33/1 -> Logical37/3
  Logical36/1 -> Logical37/4
  Logical37/1 -> Counter3/2  "gbe_dv_error"
  [clr_status] -> Counter3/1
  Counter3/1 -> gbe_valid_err/1(out_reg)
  pipeline436/1(q) -> Mux25/1
  pipeline437/1(q) -> pipeline438/1(d)
  pipeline438/1(q) -> Mux26/1
  [rampdata0] -> Mux20/2
  [sel_ramp80] -> Mux20/1
  pack_80_64_4/3(data64) -> pipeline439/1(d)
  pipeline439/1(q) -> Mux20/3
  [rampdata1] -> Mux21/2
  [sel_ramp80] -> Mux21/1
  pipeline440/1(q) -> Mux21/3
  pack_80_64_5/3(data64) -> pipeline440/1(d)  "d64_00"
  [rampdata2] -> Mux10/2
  [sel_ramp80] -> Mux10/1
  pipeline441/1(q) -> Mux10/3
  [rampdata3] -> Mux11/2
  [sel_ramp80] -> Mux11/1
  pipeline442/1(q) -> Mux11/3
  pack_80_64_7/3(data64) -> pipeline442/1(d)
  pack_80_64_6/3(data64) -> pipeline441/1(d)
  Mux10/1 -> spead_pack6/3(data64)
  Delay109/1 -> Mux12/1
  [speadtime0] -> Mux12/3
  Mux12/1 -> pack_80_64_4/1(data80)  "d80_in"
  Delay113/1 -> Mux13/1
  [speadtime1] -> Mux13/3
  Mux13/1 -> pack_80_64_5/1(data80)
  Delay117/1 -> Mux14/1
  [speadtime0] -> Mux14/3
  Mux14/1 -> pack_80_64_6/1(data80)
  pipeline348/1(q) -> Mux14/2
  Delay104/1 -> Mux15/1
  [speadtime1] -> Mux15/3
  Mux15/1 -> pack_80_64_7/1(data80)
  pipeline271/1(q) -> Mux15/2
  bus_expand3/1(msb_out4) -> Terminator23/1  "tx_d3"
  bus_expand3/2(out3) -> Terminator35/1  "tx_d2"
  bus_expand3/3(out2) -> Terminator44/1  "tx_d1"
  Constant127/1 -> Relational12/1
  Relational12/1 -> Inverter1/1
  Inverter1/1 -> Logical38/2
  [sp256_eof] -> Logical38/1
  [clr_status] -> Counter5/1
  Counter5/1 -> gbe_last_value_err/1(out_reg)
  Logical38/1 -> Counter5/2  "last_value_error"
  [sp256_data] -> bus_expand3/1(bus_in)
  [tvg_select0] -> Delay118/1
  Delay118/1 -> Gateway Out61/1, Mux22/1
  Delay119/1 -> Mux22/2
  Delay125/1 -> Mux22/3
  [tvg_pol0] -> Delay119/1
  [data_80_0] -> Delay125/1
  Mux22/1 -> Assert2/1
  [tvg_select1] -> Delay135/1
  Mux23/1 -> Assert3/1  "d80_0"
  [data_80_1] -> Delay137/1
  [tvg_pol1] -> Delay136/1
  Delay135/1 -> Mux23/1
  Delay137/1 -> Mux23/3
  Delay136/1 -> Mux23/2
  Constant187/1 -> Relational12/2
  bus_expand3/4(lsb_out1) -> Terminator55/1  "tx_d0"
  Mux27/1 -> Terminator65/1  "tx_dv"
  [gbe_txip] -> Gateway Out228/1
  Gateway Out228/1 -> To Workspace31/1
  Gateway Out239/1 -> To Workspace32/1
  Gateway Out30/1 -> To Workspace34/1
  Gateway Out31/1 -> To Workspace35/1
  Gateway Out34/1 -> To Workspace36/1
  Gateway Out35/1 -> To Workspace38/1
  Gateway Out39/1 -> To Workspace39/1
  Gateway Out41/1 -> To Workspace41/1
  Gateway Out42/1 -> To Workspace42/1
  Gateway Out29/1 -> To Workspace29/1
  Gateway Out40/1 -> To Workspace40/1
  Gateway Out62/1 -> To Workspace62/1
  Gateway Out43/1 -> To Workspace43/1
  Gateway Out44/1 -> To Workspace44/1
  Gateway Out45/1 -> To Workspace45/1
  Gateway Out46/1 -> To Workspace46/1
  [gbe_ip0] -> Gateway Out43/1, Mux17/3
  pipeline421/1(q) -> Mux18/1
  pipeline422/1(q) -> Mux19/1
  Gateway Out95/1 -> To Workspace239/1
  [spead_valid0] -> Gateway Out95/1
  Gateway Out47/1 -> To Workspace47/1
  [spead_valid1] -> Gateway Out47/1
  Gateway Out48/1 -> To Workspace48/1
  Gateway Out49/1 -> To Workspace49/1
  Gateway Out50/1 -> To Workspace50/1
  Gateway Out53/1 -> To Workspace53/1
  Gateway Out54/1 -> To Workspace54/1
  Gateway Out55/1 -> To Workspace55/1
  Gateway Out56/1 -> To Workspace56/1
  Gateway Out57/1 -> To Workspace57/1
  pipeline270/1(q) -> Gateway Out50/1, [sp256_data0]
  Gateway Out52/1 -> To Workspace52/1
  Gateway Out59/1 -> To Workspace59/1
  Gateway Out61/1 -> To Workspace61/1
  Gateway Out63/1 -> To Workspace63/1
  Assert2/1 -> Gateway Out63/1, fifo5/1(data80), fifo4/1(data80)
  [mrst] -> fifo_select1/2(rst)
  [tvg_ltime] -> fifo_select2/1(localtime)
  [mrst] -> fifo_select2/2(rst)
  Gateway Out64/1 -> To Workspace64/1
  [spead_valid2] -> Gateway Out64/1
  Gateway Out65/1 -> To Workspace65/1
  [spead_valid3] -> Gateway Out65/1
  Gateway Out66/1 -> To Workspace66/1
  [spead_eof2] -> Gateway Out66/1
  Gateway Out67/1 -> To Workspace67/1
  Gateway Out68/1 -> To Workspace68/1
  [spead_eof1] -> Gateway Out68/1
  [spead_eof3] -> Gateway Out67/1
  Gateway Out69/1 -> To Workspace69/1
  [spead_eof0] -> Gateway Out69/1
  Gateway Out70/1 -> To Workspace70/1
  Gateway Out71/1 -> To Workspace71/1
  Gateway Out72/1 -> To Workspace72/1
  Gateway Out74/1 -> To Workspace74/1
  Gateway Out75/1 -> To Workspace75/1
  Gateway Out76/1 -> To Workspace76/1
  Gateway Out77/1 -> To Workspace77/1
  Gateway Out78/1 -> To Workspace78/1
  Gateway Out79/1 -> To Workspace79/1
  Gateway Out80/1 -> To Workspace80/1
  Gateway Out81/1 -> To Workspace81/1
  Gateway Out82/1 -> To Workspace82/1
  Gateway Out83/1 -> To Workspace83/1
  Gateway Out85/1 -> To Workspace85/1
  Constant87/1 -> test_control/1(sim_1)
  Constant91/1 -> test_control/2(sim_2)
  Gateway Out88/1 -> To Workspace88/1
  Gateway Out89/1 -> To Workspace89/1
  Gateway Out90/1 -> To Workspace90/1
  Gateway Out91/1 -> To Workspace91/1
  Gateway Out92/1 -> To Workspace92/1
  Gateway Out93/1 -> To Workspace93/1
  Gateway Out107/1 -> To Workspace107/1
  bus_expand37/1(msb_out2) -> Gateway Out107/1
  Gateway Out108/1 -> To Workspace108/1
  bus_expand37/2(lsb_out1) -> Gateway Out108/1
  Gateway Out109/1 -> To Workspace109/1
  bus_expand38/1(msb_out2) -> Gateway Out109/1
  Gateway Out110/1 -> To Workspace110/1
  bus_expand38/2(lsb_out1) -> Gateway Out110/1
  Gateway Out111/1 -> To Workspace111/1
  bus_expand39/1(msb_out2) -> Gateway Out111/1
  Gateway Out112/1 -> To Workspace112/1
  bus_expand39/2(lsb_out1) -> Gateway Out112/1
  Gateway Out113/1 -> To Workspace113/1
  bus_expand35/1(msb_out2) -> Gateway Out113/1
  Gateway Out114/1 -> To Workspace114/1
  bus_expand35/2(lsb_out1) -> Gateway Out114/1
  bus_expand36/1(msb_out4) -> Gateway Out134/1, bus_expand35/1(bus_in)
  bus_expand36/2(out3) -> Gateway Out149/1, bus_expand39/1(bus_in)
  bus_expand36/3(out2) -> bus_expand38/1(bus_in), Gateway Out148/1
  bus_expand36/4(lsb_out1) -> Gateway Out147/1, bus_expand37/1(bus_in)
  [sp256_data] -> bus_expand36/1(bus_in)
  [sp256_dv] -> Counter8/2
  Counter8/1 -> Gateway Out117/1, Register4/1, Relational15/1, Relational16/1, Relational14/1
  Constant/1 -> Relational14/2, Relational16/2, Relational15/2
  Register4/1 -> Gateway Out115/1, spead_valid_count/1(out_reg)
  [mrst] -> Counter15/1, Counter14/1, Counter13/1, Register12/2, Register11/2, Register/2, Register4/2
  Register/1 -> Convert5/1
  Convert5/1 -> Gateway Out116/1, spead_valid_err_greater/1(out_reg)
  Gateway Out115/1 -> To Workspace115/1
  Gateway Out116/1 -> To Workspace116/1
  Gateway Out117/1 -> To Workspace117/1
  Gateway Out118/1 -> To Workspace118/1
  edge_detect32/1 -> Register4/3, Delay106/1, Delay62/1, Counter8/1
  Gateway Out119/1 -> To Workspace119/1
  [rdy0] -> Gateway Out119/1
  Gateway Out120/1 -> To Workspace120/1
  Gateway Out121/1 -> To Workspace121/1
  [rdy1] -> Gateway Out121/1
  Gateway Out122/1 -> To Workspace122/1
  [rdy2] -> Gateway Out122/1
  Gateway Out123/1 -> To Workspace123/1
  [rdy3] -> Gateway Out123/1
  [vld0] -> Gateway Out120/1
  Gateway Out125/1 -> To Workspace125/1
  Gateway Out126/1 -> To Workspace126/1
  Gateway Out127/1 -> To Workspace127/1
  [vld1] -> Gateway Out125/1
  [vld2] -> Gateway Out126/1
  [vld3] -> Gateway Out127/1
  Gateway Out129/1 -> To Workspace129/1
  Gateway Out134/1 -> To Workspace134/1
  Gateway Out147/1 -> To Workspace147/1
  Gateway Out148/1 -> To Workspace148/1
  Gateway Out149/1 -> To Workspace149/1
  Gateway Out58/1 -> To Workspace58/1
  munge/1(dout) -> [sp256_data]
  Register11/1 -> Convert7/1
  Convert7/1 -> spead_valid_err_less/1(out_reg), Gateway Out175/1
  Gateway Out175/1 -> To Workspace175/1
  Gateway Out180/1 -> To Workspace180/1
  Relational14/1 -> Counter13/2, Gateway Out118/1, Register/3, Register/1
  Relational16/1 -> Gateway Out187/1, Logical41/1
  Register12/1 -> Convert9/1
  Convert9/1 -> Gateway Out181/1, spead_valid_len/1(out_reg)
  Gateway Out181/1 -> To Workspace181/1
  Gateway Out182/1 -> To Workspace182/1
  Counter13/1 -> Gateway Out183/1, spead_valid_err_cnt_greater/1(out_reg)
  Counter14/1 -> Gateway Out184/1, spead_valid_err_cnt_less/1(out_reg)
  Gateway Out183/1 -> To Workspace183/1
  Gateway Out184/1 -> To Workspace184/1
  Gateway Out185/1 -> To Workspace185/1
  Counter15/1 -> Gateway Out185/1, spead_valid_len_cnt/1(out_reg)
  Logical40/1 -> Gateway Out180/1, Register11/3, Counter14/2, Register11/1
  [sp256_eof] -> edge_detect32/1
  Logical41/1 -> Counter15/2, Gateway Out182/1, Register12/3, Register12/1
  Gateway Out186/1 -> To Workspace186/1
  Relational15/1 -> Gateway Out186/1, Logical40/1
  Gateway Out187/1 -> To Workspace187/1
  Delay62/1 -> Logical40/2
  Delay106/1 -> Gateway Out188/1, Logical41/2
  Gateway Out188/1 -> To Workspace188/1
  Gateway Out213/1 -> To Workspace213/1
  [speadtime0] -> Gateway Out213/1
  Gateway Out221/1 -> To Workspace221/1
  [speadtime1] -> Gateway Out221/1
  bus_constant/1(dout) -> pipeline458/1(d)
